simulink library "ammclib_bam_S32K3xx"  (R2016a)
(part 25 of 50)

      |   if (wksi<=0)
      |     warning('Current loop attenuation must be positive.');
      |   end
      |   if (wksi>1)
      |     warning('Current loop attenuation must not exceed 1.');
      |   end
      |   if (J<=0)
      |     warning('Moment of inertia J must be positive.');
      |   end
      |   if (Kt<=0)
      |     warning('Torque constant Kt must be positive.');
      |   end
      |   if (lambdaW<0)
      |     warning('MA filter smoothing factor must be in the range 0..1.');
      |   end
      |   if (lambdaW>1)
      |     warning('MA filter smoothing factor must be in the range 0..1.');
      |   end
      |   if (lambdaFW<0)
      |     warning('MA filter smoothing factor must be in the range 0..1.');
      |   end
      |   if (lambdaFW>1)
      |     warning('MA filter smoothing factor must be in the range 0..1.');
      |   end
      |   if (udcbus<=0)
      |     warning('DC bus voltage must be positive.');
      |   end
      |   if (imax<=0)
      |     warning('Max. phase current must be positive.');
      |   end
      |   if (mechspeed<=0)
      |     warning('Max. speed must be positive.');
      |   end
      |   if (polepairs<1)
      |     warning('Number of pole pairs must be a natural number (1, 2, 3, ...).');
      |   end
      |   if (round(polepairs)~=polepairs)
      |     warning('Number of pole pairs must be a natural number (1, 2, 3, ...).');
      |   end
      |   w0=6.283185307179586*wf0;
      |   pgain=2.0*wksi*w0*J/Kt;
      |   igain=w0*w0*J/Kt;
      |   wmax=polepairs*mechspeed*0.1047197551196598;
      |   fltPropGainQ=pgain;
      |   fltIntegGainQ=igain*SampleTime*0.5;
      |   fltLowerLimitQ=-wmax;
      |   fltUpperLimitQ=wmax;
      |   fltPropGainFW=0.9*pgain;
      |   fltIntegGainFW=fltIntegGainQ;
      |   if (Idmax<0)
      |     iratio=Idmax/imax;
      |     iratio=abs(iratio);
      |     if (abs(iratio) > 1)
      |       iratio = 0;
      |     end
      |     lowlim=acos(iratio)-1.570796326794897;
      |   else
      |     lowlim=0.0;
      |   end
      |   fltLowerLimitFW=lowlim;
      |   fltUpperLimitFW=0.0;
      |   fltLambdaW=lambdaW;
      |   fltLambdaFW=lambdaFW;
      |   rampsc=polepairs*abs(ramprpm)*0.1047197551196598;
      |   fltRampUp=rampsc;
      |   fltRampDown=rampsc;
      |   fltUmaxDivImax=0.5773502691896258*udcbus/imax;
      |   if isnan(fltUmaxDivImax)
      |     if ~strcmp(fltUmaxDivImax_bkup,'0')
      |       set_param(gcb,'fltUmaxDivImax','0');
      |     end
      |   else
      |     tmps=num2str(fltUmaxDivImax);
      |     if ~strcmp(fltUmaxDivImax_bkup,tmps)
      |       set_param(gcb,'fltUmaxDivImax',tmps);
      |     end
      |   end
      |   if isnan(fltLambdaW)
      |     if ~strcmp(fltLambdaW_bkup,'0')
      |       set_param(gcb,'fltLambdaW','0');
      |     end
      |   else
      |     tmps=num2str(fltLambdaW);
      |     if ~strcmp(fltLambdaW_bkup,tmps)
      |       set_param(gcb,'fltLambdaW',tmps);
      |     end
      |   end
      |   if isnan(fltLambdaFW)
      |     if ~strcmp(fltLambdaFW_bkup,'0')
      |       set_param(gcb,'fltLambdaFW','0');
      |     end
      |   else
      |     tmps=num2str(fltLambdaFW);
      |     if ~strcmp(fltLambdaFW_bkup,tmps)
      |       set_param(gcb,'fltLambdaFW',tmps);
      |     end
      |   end
      |   if isnan(fltPropGainQ)
      |     if ~strcmp(fltPropGainQ_bkup,'0')
      |       set_param(gcb,'fltPropGainQ','0');
      |     end
      |   else
      |     tmps=num2str(fltPropGainQ);
      |     if ~strcmp(fltPropGainQ_bkup,tmps)
      |       set_param(gcb,'fltPropGainQ',tmps);
      |     end
      |   end
      |   if isnan(fltIntegGainQ)
      |     if ~strcmp(fltIntegGainQ_bkup,'0')
      |       set_param(gcb,'fltIntegGainQ','0');
      |     end
      |   else
      |     tmps=num2str(fltIntegGainQ);
      |     if ~strcmp(fltIntegGainQ_bkup,tmps)
      |       set_param(gcb,'fltIntegGainQ',tmps);
      |     end
      |   end
      |   if isnan(fltLowerLimitQ)
      |     if ~strcmp(fltLowerLimitQ_bkup,'0')
      |       set_param(gcb,'fltLowerLimitQ','0');
      |     end
      |   else
      |     tmps=num2str(fltLowerLimitQ);
      |     if ~strcmp(fltLowerLimitQ_bkup,tmps)
      |       set_param(gcb,'fltLowerLimitQ',tmps);
      |     end
      |   end
      |   if isnan(fltUpperLimitQ)
      |     if ~strcmp(fltUpperLimitQ_bkup,'0')
      |       set_param(gcb,'fltUpperLimitQ','0');
      |     end
      |   else
      |     tmps=num2str(fltUpperLimitQ);
      |     if ~strcmp(fltUpperLimitQ_bkup,tmps)
      |       set_param(gcb,'fltUpperLimitQ',tmps);
      |     end
      |   end
      |   if isnan(fltPropGainFW)
      |     if ~strcmp(fltPropGainFW_bkup,'0')
      |       set_param(gcb,'fltPropGainFW','0');
      |     end
      |   else
      |     tmps=num2str(fltPropGainFW);
      |     if ~strcmp(fltPropGainFW_bkup,tmps)
      |       set_param(gcb,'fltPropGainFW',tmps);
      |     end
      |   end
      |   if isnan(fltIntegGainFW)
      |     if ~strcmp(fltIntegGainFW_bkup,'0')
      |       set_param(gcb,'fltIntegGainFW','0');
      |     end
      |   else
      |     tmps=num2str(fltIntegGainFW);
      |     if ~strcmp(fltIntegGainFW_bkup,tmps)
      |       set_param(gcb,'fltIntegGainFW',tmps);
      |     end
      |   end
      |   if isnan(fltLowerLimitFW)
      |     if ~strcmp(fltLowerLimitFW_bkup,'0')
      |       set_param(gcb,'fltLowerLimitFW','0');
      |     end
      |   else
      |     tmps=num2str(fltLowerLimitFW);
      |     if ~strcmp(fltLowerLimitFW_bkup,tmps)
      |       set_param(gcb,'fltLowerLimitFW',tmps);
      |     end
      |   end
      |   if isnan(fltUpperLimitFW)
      |     if ~strcmp(fltUpperLimitFW_bkup,'0')
      |       set_param(gcb,'fltUpperLimitFW','0');
      |     end
      |   else
      |     tmps=num2str(fltUpperLimitFW);
      |     if ~strcmp(fltUpperLimitFW_bkup,tmps)
      |       set_param(gcb,'fltUpperLimitFW',tmps);
      |     end
      |   end
      |   if isnan(fltRampUp)
      |     if ~strcmp(fltRampUp_bkup,'0')
      |       set_param(gcb,'fltRampUp','0');
      |     end
      |   else
      |     tmps=num2str(fltRampUp);
      |     if ~strcmp(fltRampUp_bkup,tmps)
      |       set_param(gcb,'fltRampUp',tmps);
      |     end
      |   end
      |   if isnan(fltRampDown)
      |     if ~strcmp(fltRampDown_bkup,'0')
      |       set_param(gcb,'fltRampDown','0');
      |     end
      |   else
      |     tmps=num2str(fltRampDown);
      |     if ~strcmp(fltRampDown_bkup,tmps)
      |       set_param(gcb,'fltRampDown',tmps);
      |     end
      |   end
      | end
      mask Callback polepairs:
      | autoCalcEn=get_param(gcb,'autoCalcEn');
      | if strcmp(autoCalcEn,'on')
      |   SampleTime=Simulink.data.evalinGlobal(bdroot,get_param(gcb,'SampleTime'));
      |   if (SampleTime==-1)
      |     SampleTime=str2double(get_param(gcb,'SampleTime_1'));
      |   end
      |   fltUmaxDivImax_bkup=get_param(gcb,'fltUmaxDivImax');
      |   fltLambdaW_bkup=get_param(gcb,'fltLambdaW');
      |   fltLambdaFW_bkup=get_param(gcb,'fltLambdaFW');
      |   fltPropGainQ_bkup=get_param(gcb,'fltPropGainQ');
      |   fltIntegGainQ_bkup=get_param(gcb,'fltIntegGainQ');
      |   fltLowerLimitQ_bkup=get_param(gcb,'fltLowerLimitQ');
      |   fltUpperLimitQ_bkup=get_param(gcb,'fltUpperLimitQ');
      |   fltPropGainFW_bkup=get_param(gcb,'fltPropGainFW');
      |   fltIntegGainFW_bkup=get_param(gcb,'fltIntegGainFW');
      |   fltLowerLimitFW_bkup=get_param(gcb,'fltLowerLimitFW');
      |   fltUpperLimitFW_bkup=get_param(gcb,'fltUpperLimitFW');
      |   fltRampUp_bkup=get_param(gcb,'fltRampUp');
      |   fltRampDown_bkup=get_param(gcb,'fltRampDown');
      |   wf0=Simulink.data.evalinGlobal(bdroot,get_param(gcb,'wf0'));
      |   wksi=Simulink.data.evalinGlobal(bdroot,get_param(gcb,'wksi'));
      |   J=Simulink.data.evalinGlobal(bdroot,get_param(gcb,'J'));
      |   Kt=Simulink.data.evalinGlobal(bdroot,get_param(gcb,'Kt'));
      |   lambdaW=Simulink.data.evalinGlobal(bdroot,get_param(gcb,'lambdaW'));
      |   lambdaFW=Simulink.data.evalinGlobal(bdroot,get_param(gcb,'lambdaFW'));
      |   Idmax=Simulink.data.evalinGlobal(bdroot,get_param(gcb,'Idmax'));
      |   imax=Simulink.data.evalinGlobal(bdroot,get_param(gcb,'imax'));
      |   udcbus=Simulink.data.evalinGlobal(bdroot,get_param(gcb,'udcbus'));
      |   ramprpm=Simulink.data.evalinGlobal(bdroot,get_param(gcb,'ramprpm'));
      |   mechspeed=Simulink.data.evalinGlobal(bdroot,get_param(gcb,'mechspeed'));
      |   polepairs=Simulink.data.evalinGlobal(bdroot,get_param(gcb,'polepairs'));
      |   if (wf0<=0)
      |     warning('Natural frequency f0 must be positive.');
      |   end
      |   if (wksi<=0)
      |     warning('Current loop attenuation must be positive.');
      |   end
      |   if (wksi>1)
      |     warning('Current loop attenuation must not exceed 1.');
      |   end
      |   if (J<=0)
      |     warning('Moment of inertia J must be positive.');
      |   end
      |   if (Kt<=0)
      |     warning('Torque constant Kt must be positive.');
      |   end
      |   if (lambdaW<0)
      |     warning('MA filter smoothing factor must be in the range 0..1.');
      |   end
      |   if (lambdaW>1)
      |     warning('MA filter smoothing factor must be in the range 0..1.');
      |   end
      |   if (lambdaFW<0)
      |     warning('MA filter smoothing factor must be in the range 0..1.');
      |   end
      |   if (lambdaFW>1)
      |     warning('MA filter smoothing factor must be in the range 0..1.');
      |   end
      |   if (udcbus<=0)
      |     warning('DC bus voltage must be positive.');
      |   end
      |   if (imax<=0)
      |     warning('Max. phase current must be positive.');
      |   end
      |   if (mechspeed<=0)
      |     warning('Max. speed must be positive.');
      |   end
      |   if (polepairs<1)
      |     warning('Number of pole pairs must be a natural number (1, 2, 3, ...).');
      |   end
      |   if (round(polepairs)~=polepairs)
      |     warning('Number of pole pairs must be a natural number (1, 2, 3, ...).');
      |   end
      |   w0=6.283185307179586*wf0;
      |   pgain=2.0*wksi*w0*J/Kt;
      |   igain=w0*w0*J/Kt;
      |   wmax=polepairs*mechspeed*0.1047197551196598;
      |   fltPropGainQ=pgain;
      |   fltIntegGainQ=igain*SampleTime*0.5;
      |   fltLowerLimitQ=-wmax;
      |   fltUpperLimitQ=wmax;
      |   fltPropGainFW=0.9*pgain;
      |   fltIntegGainFW=fltIntegGainQ;
      |   if (Idmax<0)
      |     iratio=Idmax/imax;
      |     iratio=abs(iratio);
      |     if (abs(iratio) > 1)
      |       iratio = 0;
      |     end
      |     lowlim=acos(iratio)-1.570796326794897;
      |   else
      |     lowlim=0.0;
      |   end
      |   fltLowerLimitFW=lowlim;
      |   fltUpperLimitFW=0.0;
      |   fltLambdaW=lambdaW;
      |   fltLambdaFW=lambdaFW;
      |   rampsc=polepairs*abs(ramprpm)*0.1047197551196598;
      |   fltRampUp=rampsc;
      |   fltRampDown=rampsc;
      |   fltUmaxDivImax=0.5773502691896258*udcbus/imax;
      |   if isnan(fltUmaxDivImax)
      |     if ~strcmp(fltUmaxDivImax_bkup,'0')
      |       set_param(gcb,'fltUmaxDivImax','0');
      |     end
      |   else
      |     tmps=num2str(fltUmaxDivImax);
      |     if ~strcmp(fltUmaxDivImax_bkup,tmps)
      |       set_param(gcb,'fltUmaxDivImax',tmps);
      |     end
      |   end
      |   if isnan(fltLambdaW)
      |     if ~strcmp(fltLambdaW_bkup,'0')
      |       set_param(gcb,'fltLambdaW','0');
      |     end
      |   else
      |     tmps=num2str(fltLambdaW);
      |     if ~strcmp(fltLambdaW_bkup,tmps)
      |       set_param(gcb,'fltLambdaW',tmps);
      |     end
      |   end
      |   if isnan(fltLambdaFW)
      |     if ~strcmp(fltLambdaFW_bkup,'0')
      |       set_param(gcb,'fltLambdaFW','0');
      |     end
      |   else
      |     tmps=num2str(fltLambdaFW);
      |     if ~strcmp(fltLambdaFW_bkup,tmps)
      |       set_param(gcb,'fltLambdaFW',tmps);
      |     end
      |   end
      |   if isnan(fltPropGainQ)
      |     if ~strcmp(fltPropGainQ_bkup,'0')
      |       set_param(gcb,'fltPropGainQ','0');
      |     end
      |   else
      |     tmps=num2str(fltPropGainQ);
      |     if ~strcmp(fltPropGainQ_bkup,tmps)
      |       set_param(gcb,'fltPropGainQ',tmps);
      |     end
      |   end
      |   if isnan(fltIntegGainQ)
      |     if ~strcmp(fltIntegGainQ_bkup,'0')
      |       set_param(gcb,'fltIntegGainQ','0');
      |     end
      |   else
      |     tmps=num2str(fltIntegGainQ);
      |     if ~strcmp(fltIntegGainQ_bkup,tmps)
      |       set_param(gcb,'fltIntegGainQ',tmps);
      |     end
      |   end
      |   if isnan(fltLowerLimitQ)
      |     if ~strcmp(fltLowerLimitQ_bkup,'0')
      |       set_param(gcb,'fltLowerLimitQ','0');
      |     end
      |   else
      |     tmps=num2str(fltLowerLimitQ);
      |     if ~strcmp(fltLowerLimitQ_bkup,tmps)
      |       set_param(gcb,'fltLowerLimitQ',tmps);
      |     end
      |   end
      |   if isnan(fltUpperLimitQ)
      |     if ~strcmp(fltUpperLimitQ_bkup,'0')
      |       set_param(gcb,'fltUpperLimitQ','0');
      |     end
      |   else
      |     tmps=num2str(fltUpperLimitQ);
      |     if ~strcmp(fltUpperLimitQ_bkup,tmps)
      |       set_param(gcb,'fltUpperLimitQ',tmps);
      |     end
      |   end
      |   if isnan(fltPropGainFW)
      |     if ~strcmp(fltPropGainFW_bkup,'0')
      |       set_param(gcb,'fltPropGainFW','0');
      |     end
      |   else
      |     tmps=num2str(fltPropGainFW);
      |     if ~strcmp(fltPropGainFW_bkup,tmps)
      |       set_param(gcb,'fltPropGainFW',tmps);
      |     end
      |   end
      |   if isnan(fltIntegGainFW)
      |     if ~strcmp(fltIntegGainFW_bkup,'0')
      |       set_param(gcb,'fltIntegGainFW','0');
      |     end
      |   else
      |     tmps=num2str(fltIntegGainFW);
      |     if ~strcmp(fltIntegGainFW_bkup,tmps)
      |       set_param(gcb,'fltIntegGainFW',tmps);
      |     end
      |   end
      |   if isnan(fltLowerLimitFW)
      |     if ~strcmp(fltLowerLimitFW_bkup,'0')
      |       set_param(gcb,'fltLowerLimitFW','0');
      |     end
      |   else
      |     tmps=num2str(fltLowerLimitFW);
      |     if ~strcmp(fltLowerLimitFW_bkup,tmps)
      |       set_param(gcb,'fltLowerLimitFW',tmps);
      |     end
      |   end
      |   if isnan(fltUpperLimitFW)
      |     if ~strcmp(fltUpperLimitFW_bkup,'0')
      |       set_param(gcb,'fltUpperLimitFW','0');
      |     end
      |   else
      |     tmps=num2str(fltUpperLimitFW);
      |     if ~strcmp(fltUpperLimitFW_bkup,tmps)
      |       set_param(gcb,'fltUpperLimitFW',tmps);
      |     end
      |   end
      |   if isnan(fltRampUp)
      |     if ~strcmp(fltRampUp_bkup,'0')
      |       set_param(gcb,'fltRampUp','0');
      |     end
      |   else
      |     tmps=num2str(fltRampUp);
      |     if ~strcmp(fltRampUp_bkup,tmps)
      |       set_param(gcb,'fltRampUp',tmps);
      |     end
      |   end
      |   if isnan(fltRampDown)
      |     if ~strcmp(fltRampDown_bkup,'0')
      |       set_param(gcb,'fltRampDown','0');
      |     end
      |   else
      |     tmps=num2str(fltRampDown);
      |     if ~strcmp(fltRampDown_bkup,tmps)
      |       set_param(gcb,'fltRampDown',tmps);
      |     end
      |   end
      | end
      mask Callback autoCalcEn:
      | maskStr=get_param(gcb,'showStates');
      | if strcmp(maskStr,'Hide (faster execution)')
      |   p=Simulink.Mask.get(gcb);
      |   autoCalcEn=get_param(gcb,'autoCalcEn');
      |   hintText=p.getDialogControl('timeHint');
      |   if strcmp(autoCalcEn,'on')
      |     param=p.getParameter('polepairs');
      |     if strcmp(param.Enabled,'off')
      |       SampleTime=Simulink.data.evalinGlobal(bdroot,get_param(gcb,'SampleTime'));
      |       if SampleTime==-1
      |         SampleTime=str2double(get_param(gcb,'SampleTime_1'));
      |         if isnan(SampleTime)
      |           hintText.Prompt=['Note: Implementation parameters cannot be calculated yet because the block''s inherited sample time is unknown. Simulink will update the sample time when you run the simulation.'];
      |         else
      |           hintText.Prompt=['Caution: Implementation parameters depend on inherited sample time. Make sure that the sample time of the block''s inputs corresponds to the sampling period in the target application.'];
      |         end
      |       else
      |         hintText.Prompt='Caution: Implementation parameters depend on the sample time. Make sure that the simulation time step corresponds to the sampling period in the target application.';
      |       end
      |       p=Simulink.Mask.get(gcb);
      |       param=p.getParameter('wf0');
      |       param.set('Enabled','on');
      |       param=p.getParameter('wksi');
      |       param.set('Enabled','on');
      |       param=p.getParameter('J');
      |       param.set('Enabled','on');
      |       param=p.getParameter('Kt');
      |       param.set('Enabled','on');
      |       param=p.getParameter('lambdaW');
      |       param.set('Enabled','on');
      |       param=p.getParameter('lambdaFW');
      |       param.set('Enabled','on');
      |       param=p.getParameter('Idmax');
      |       param.set('Enabled','on');
      |       param=p.getParameter('imax');
      |       param.set('Enabled','on');
      |       param=p.getParameter('udcbus');
      |       param.set('Enabled','on');
      |       param=p.getParameter('ramprpm');
      |       param.set('Enabled','on');
      |       param=p.getParameter('mechspeed');
      |       param.set('Enabled','on');
      |       param=p.getParameter('polepairs');
      |       param.set('Enabled','on');
      |     else
      |       SampleTime=Simulink.data.evalinGlobal(bdroot,get_param(gcb,'SampleTime'));
      |       if SampleTime==-1
      |         SampleTime=str2double(get_param(gcb,'SampleTime_1'));
      |       end
      |     end
      |     fltUmaxDivImax_bkup=get_param(gcb,'fltUmaxDivImax');
      |     fltLambdaW_bkup=get_param(gcb,'fltLambdaW');
      |     fltLambdaFW_bkup=get_param(gcb,'fltLambdaFW');
      |     fltPropGainQ_bkup=get_param(gcb,'fltPropGainQ');
      |     fltIntegGainQ_bkup=get_param(gcb,'fltIntegGainQ');
      |     fltLowerLimitQ_bkup=get_param(gcb,'fltLowerLimitQ');
      |     fltUpperLimitQ_bkup=get_param(gcb,'fltUpperLimitQ');
      |     fltPropGainFW_bkup=get_param(gcb,'fltPropGainFW');
      |     fltIntegGainFW_bkup=get_param(gcb,'fltIntegGainFW');
      |     fltLowerLimitFW_bkup=get_param(gcb,'fltLowerLimitFW');
      |     fltUpperLimitFW_bkup=get_param(gcb,'fltUpperLimitFW');
      |     fltRampUp_bkup=get_param(gcb,'fltRampUp');
      |     fltRampDown_bkup=get_param(gcb,'fltRampDown');
      |     wf0=Simulink.data.evalinGlobal(bdroot,get_param(gcb,'wf0'));
      |     wksi=Simulink.data.evalinGlobal(bdroot,get_param(gcb,'wksi'));
      |     J=Simulink.data.evalinGlobal(bdroot,get_param(gcb,'J'));
      |     Kt=Simulink.data.evalinGlobal(bdroot,get_param(gcb,'Kt'));
      |     lambdaW=Simulink.data.evalinGlobal(bdroot,get_param(gcb,'lambdaW'));
      |     lambdaFW=Simulink.data.evalinGlobal(bdroot,get_param(gcb,'lambdaFW'));
      |     Idmax=Simulink.data.evalinGlobal(bdroot,get_param(gcb,'Idmax'));
      |     imax=Simulink.data.evalinGlobal(bdroot,get_param(gcb,'imax'));
      |     udcbus=Simulink.data.evalinGlobal(bdroot,get_param(gcb,'udcbus'));
      |     ramprpm=Simulink.data.evalinGlobal(bdroot,get_param(gcb,'ramprpm'));
      |     mechspeed=Simulink.data.evalinGlobal(bdroot,get_param(gcb,'mechspeed'));
      |     polepairs=Simulink.data.evalinGlobal(bdroot,get_param(gcb,'polepairs'));
      |     if (wf0<=0)
      |       warning('Natural frequency f0 must be positive.');
      |     end
      |     if (wksi<=0)
      |       warning('Current loop attenuation must be positive.');
      |     end
      |     if (wksi>1)
      |       warning('Current loop attenuation must not exceed 1.');
      |     end
      |     if (J<=0)
      |       warning('Moment of inertia J must be positive.');
      |     end
      |     if (Kt<=0)
      |       warning('Torque constant Kt must be positive.');
      |     end
      |     if (lambdaW<0)
      |       warning('MA filter smoothing factor must be in the range 0..1.');
      |     end
      |     if (lambdaW>1)
      |       warning('MA filter smoothing factor must be in the range 0..1.');
      |     end
      |     if (lambdaFW<0)
      |       warning('MA filter smoothing factor must be in the range 0..1.');
      |     end
      |     if (lambdaFW>1)
      |       warning('MA filter smoothing factor must be in the range 0..1.');
      |     end
      |     if (udcbus<=0)
      |       warning('DC bus voltage must be positive.');
      |     end
      |     if (imax<=0)
      |       warning('Max. phase current must be positive.');
      |     end
      |     if (mechspeed<=0)
      |       warning('Max. speed must be positive.');
      |     end
      |     if (polepairs<1)
      |       warning('Number of pole pairs must be a natural number (1, 2, 3, ...).');
      |     end
      |     if (round(polepairs)~=polepairs)
      |       warning('Number of pole pairs must be a natural number (1, 2, 3, ...).');
      |     end
      |     w0=6.283185307179586*wf0;
      |     pgain=2.0*wksi*w0*J/Kt;
      |     igain=w0*w0*J/Kt;
      |     wmax=polepairs*mechspeed*0.1047197551196598;
      |     fltPropGainQ=pgain;
      |     fltIntegGainQ=igain*SampleTime*0.5;
      |     fltLowerLimitQ=-wmax;
      |     fltUpperLimitQ=wmax;
      |     fltPropGainFW=0.9*pgain;
      |     fltIntegGainFW=fltIntegGainQ;
      |     if (Idmax<0)
      |       iratio=Idmax/imax;
      |       iratio=abs(iratio);
      |       if (abs(iratio) > 1)
      |         iratio = 0;
      |       end
      |       lowlim=acos(iratio)-1.570796326794897;
      |     else
      |       lowlim=0.0;
      |     end
      |     fltLowerLimitFW=lowlim;
      |     fltUpperLimitFW=0.0;
      |     fltLambdaW=lambdaW;
      |     fltLambdaFW=lambdaFW;
      |     rampsc=polepairs*abs(ramprpm)*0.1047197551196598;
      |     fltRampUp=rampsc;
      |     fltRampDown=rampsc;
      |     fltUmaxDivImax=0.5773502691896258*udcbus/imax;
      |     if isnan(fltUmaxDivImax)
      |       if ~strcmp(fltUmaxDivImax_bkup,'0')
      |         set_param(gcb,'fltUmaxDivImax','0');
      |       end
      |     else
      |       tmps=num2str(fltUmaxDivImax);
      |       if ~strcmp(fltUmaxDivImax_bkup,tmps)
      |         set_param(gcb,'fltUmaxDivImax',tmps);
      |       end
      |     end
      |     if isnan(fltLambdaW)
      |       if ~strcmp(fltLambdaW_bkup,'0')
      |         set_param(gcb,'fltLambdaW','0');
      |       end
      |     else
      |       tmps=num2str(fltLambdaW);
      |       if ~strcmp(fltLambdaW_bkup,tmps)
      |         set_param(gcb,'fltLambdaW',tmps);
      |       end
      |     end
      |     if isnan(fltLambdaFW)
      |       if ~strcmp(fltLambdaFW_bkup,'0')
      |         set_param(gcb,'fltLambdaFW','0');
      |       end
      |     else
      |       tmps=num2str(fltLambdaFW);
      |       if ~strcmp(fltLambdaFW_bkup,tmps)
      |         set_param(gcb,'fltLambdaFW',tmps);
      |       end
      |     end
      |     if isnan(fltPropGainQ)
      |       if ~strcmp(fltPropGainQ_bkup,'0')
      |         set_param(gcb,'fltPropGainQ','0');
      |       end
      |     else
      |       tmps=num2str(fltPropGainQ);
      |       if ~strcmp(fltPropGainQ_bkup,tmps)
      |         set_param(gcb,'fltPropGainQ',tmps);
      |       end
      |     end
      |     if isnan(fltIntegGainQ)
      |       if ~strcmp(fltIntegGainQ_bkup,'0')
      |         set_param(gcb,'fltIntegGainQ','0');
      |       end
      |     else
      |       tmps=num2str(fltIntegGainQ);
      |       if ~strcmp(fltIntegGainQ_bkup,tmps)
      |         set_param(gcb,'fltIntegGainQ',tmps);
      |       end
      |     end
      |     if isnan(fltLowerLimitQ)
      |       if ~strcmp(fltLowerLimitQ_bkup,'0')
      |         set_param(gcb,'fltLowerLimitQ','0');
      |       end
      |     else
      |       tmps=num2str(fltLowerLimitQ);
      |       if ~strcmp(fltLowerLimitQ_bkup,tmps)
      |         set_param(gcb,'fltLowerLimitQ',tmps);
      |       end
      |     end
      |     if isnan(fltUpperLimitQ)
      |       if ~strcmp(fltUpperLimitQ_bkup,'0')
      |         set_param(gcb,'fltUpperLimitQ','0');
      |       end
      |     else
      |       tmps=num2str(fltUpperLimitQ);
      |       if ~strcmp(fltUpperLimitQ_bkup,tmps)
      |         set_param(gcb,'fltUpperLimitQ',tmps);
      |       end
      |     end
      |     if isnan(fltPropGainFW)
      |       if ~strcmp(fltPropGainFW_bkup,'0')
      |         set_param(gcb,'fltPropGainFW','0');
      |       end
      |     else
      |       tmps=num2str(fltPropGainFW);
      |       if ~strcmp(fltPropGainFW_bkup,tmps)
      |         set_param(gcb,'fltPropGainFW',tmps);
      |       end
      |     end
      |     if isnan(fltIntegGainFW)
      |       if ~strcmp(fltIntegGainFW_bkup,'0')
      |         set_param(gcb,'fltIntegGainFW','0');
      |       end
      |     else
      |       tmps=num2str(fltIntegGainFW);
      |       if ~strcmp(fltIntegGainFW_bkup,tmps)
      |         set_param(gcb,'fltIntegGainFW',tmps);
      |       end
      |     end
      |     if isnan(fltLowerLimitFW)
      |       if ~strcmp(fltLowerLimitFW_bkup,'0')
      |         set_param(gcb,'fltLowerLimitFW','0');
      |       end
      |     else
      |       tmps=num2str(fltLowerLimitFW);
      |       if ~strcmp(fltLowerLimitFW_bkup,tmps)
      |         set_param(gcb,'fltLowerLimitFW',tmps);
      |       end
      |     end
      |     if isnan(fltUpperLimitFW)
      |       if ~strcmp(fltUpperLimitFW_bkup,'0')
      |         set_param(gcb,'fltUpperLimitFW','0');
      |       end
      |     else
      |       tmps=num2str(fltUpperLimitFW);
      |       if ~strcmp(fltUpperLimitFW_bkup,tmps)
      |         set_param(gcb,'fltUpperLimitFW',tmps);
      |       end
      |     end
      |     if isnan(fltRampUp)
      |       if ~strcmp(fltRampUp_bkup,'0')
      |         set_param(gcb,'fltRampUp','0');
      |       end
      |     else
      |       tmps=num2str(fltRampUp);
      |       if ~strcmp(fltRampUp_bkup,tmps)
      |         set_param(gcb,'fltRampUp',tmps);
      |       end
      |     end
      |     if isnan(fltRampDown)
      |       if ~strcmp(fltRampDown_bkup,'0')
      |         set_param(gcb,'fltRampDown','0');
      |       end
      |     else
      |       tmps=num2str(fltRampDown);
      |       if ~strcmp(fltRampDown_bkup,tmps)
      |         set_param(gcb,'fltRampDown',tmps);
      |       end
      |     end
      |   else
      |     param=p.getParameter('polepairs');
      |     if strcmp(param.Enabled,'on')
      |       hintText.Prompt='Caution: Implementation parameters are fixed.';
      |       p=Simulink.Mask.get(gcb);
      |       param=p.getParameter('wf0');
      |       param.set('Enabled','off');
      |       param=p.getParameter('wksi');
      |       param.set('Enabled','off');
      |       param=p.getParameter('J');
      |       param.set('Enabled','off');
      |       param=p.getParameter('Kt');
      |       param.set('Enabled','off');
      |       param=p.getParameter('lambdaW');
      |       param.set('Enabled','off');
      |       param=p.getParameter('lambdaFW');
      |       param.set('Enabled','off');
      |       param=p.getParameter('Idmax');
      |       param.set('Enabled','off');
      |       param=p.getParameter('imax');
      |       param.set('Enabled','off');
      |       param=p.getParameter('udcbus');
      |       param.set('Enabled','off');
      |       param=p.getParameter('ramprpm');
      |       param.set('Enabled','off');
      |       param=p.getParameter('mechspeed');
      |       param.set('Enabled','off');
      |       param=p.getParameter('polepairs');
      |       param.set('Enabled','off');
      |     end
      |   end
      | end
      mask DialogControl CompBut Prompt: Recalculate sample times
      mask DialogControl CompBut Tooltip: Simulink updates the sample times of all blocks when the simulation is run. This button will update the sample times now.
      mask DialogControl CompBut Callback:
      | btn=questdlg('This will apply all changes in all open dialog boxes and update the schematic. Do you want to proceed?','Apply all changes','Continue','Cancel','Continue');
      | if strcmp(btn,'Continue')
      |   dlgs=DAStudio.ToolRoot.getOpenDialogs;
      |   for i=1:length(dlgs)
      |     dlgs(i).apply;
      |   end
      |   try
      |     SampleTime_1=str2double(get_param(gcb,'SampleTime_1'));
      |     ts=Simulink.Block.getSampleTimes(gcb);
      |     ts=ts(1).Value(1);
      |     if (SampleTime_1 ~= ts)
      |       SampleTime_1=ts;
      |       set_param(gcb,'SampleTime_1',num2str(ts));
      |       autoCalcEn=get_param(gcb,'autoCalcEn');
      |       if strcmp(autoCalcEn,'on')
      |         SampleTime=Simulink.data.evalinGlobal(bdroot,get_param(gcb,'SampleTime'));
      |         p=Simulink.Mask.get(gcb);
      |         hintText=p.getDialogControl('timeHint');
      |         if SampleTime==-1
      |           SampleTime=SampleTime_1;
      |           hintText.Prompt='Caution: Implementation parameters depend on inherited sample time. Make sure that the sample time of the block''s inputs corresponds to the sampling period in the target application.';
      |         else
      |           hintText.Prompt='Caution: Implementation parameters depend on the sample time. Make sure that the simulation time step corresponds to the sampling period in the target application.';
      |         end
      |         fltUmaxDivImax_bkup=get_param(gcb,'fltUmaxDivImax');
      |         fltLambdaW_bkup=get_param(gcb,'fltLambdaW');
      |         fltLambdaFW_bkup=get_param(gcb,'fltLambdaFW');
      |         fltPropGainQ_bkup=get_param(gcb,'fltPropGainQ');
      |         fltIntegGainQ_bkup=get_param(gcb,'fltIntegGainQ');
      |         fltLowerLimitQ_bkup=get_param(gcb,'fltLowerLimitQ');
      |         fltUpperLimitQ_bkup=get_param(gcb,'fltUpperLimitQ');
      |         fltPropGainFW_bkup=get_param(gcb,'fltPropGainFW');
      |         fltIntegGainFW_bkup=get_param(gcb,'fltIntegGainFW');
      |         fltLowerLimitFW_bkup=get_param(gcb,'fltLowerLimitFW');
      |         fltUpperLimitFW_bkup=get_param(gcb,'fltUpperLimitFW');
      |         fltRampUp_bkup=get_param(gcb,'fltRampUp');
      |         fltRampDown_bkup=get_param(gcb,'fltRampDown');
      |         wf0=Simulink.data.evalinGlobal(bdroot,get_param(gcb,'wf0'));
      |         wksi=Simulink.data.evalinGlobal(bdroot,get_param(gcb,'wksi'));
      |         J=Simulink.data.evalinGlobal(bdroot,get_param(gcb,'J'));
      |         Kt=Simulink.data.evalinGlobal(bdroot,get_param(gcb,'Kt'));
      |         lambdaW=Simulink.data.evalinGlobal(bdroot,get_param(gcb,'lambdaW'));
      |         lambdaFW=Simulink.data.evalinGlobal(bdroot,get_param(gcb,'lambdaFW'));
      |         Idmax=Simulink.data.evalinGlobal(bdroot,get_param(gcb,'Idmax'));
      |         imax=Simulink.data.evalinGlobal(bdroot,get_param(gcb,'imax'));
      |         udcbus=Simulink.data.evalinGlobal(bdroot,get_param(gcb,'udcbus'));
      |         ramprpm=Simulink.data.evalinGlobal(bdroot,get_param(gcb,'ramprpm'));
      |         mechspeed=Simulink.data.evalinGlobal(bdroot,get_param(gcb,'mechspeed'));
      |         polepairs=Simulink.data.evalinGlobal(bdroot,get_param(gcb,'polepairs'));
      |         if (wf0<=0)
      |           warning('Natural frequency f0 must be positive.');
      |         end
      |         if (wksi<=0)
      |           warning('Current loop attenuation must be positive.');
      |         end
      |         if (wksi>1)
      |           warning('Current loop attenuation must not exceed 1.');
      |         end
      |         if (J<=0)
      |           warning('Moment of inertia J must be positive.');
      |         end
      |         if (Kt<=0)
      |           warning('Torque constant Kt must be positive.');
      |         end
      |         if (lambdaW<0)
      |           warning('MA filter smoothing factor must be in the range 0..1.');
      |         end
      |         if (lambdaW>1)
      |           warning('MA filter smoothing factor must be in the range 0..1.');
      |         end
      |         if (lambdaFW<0)
      |           warning('MA filter smoothing factor must be in the range 0..1.');
      |         end
      |         if (lambdaFW>1)
      |           warning('MA filter smoothing factor must be in the range 0..1.');
      |         end
      |         if (udcbus<=0)
      |           warning('DC bus voltage must be positive.');
      |         end
      |         if (imax<=0)
      |           warning('Max. phase current must be positive.');
      |         end
      |         if (mechspeed<=0)
      |           warning('Max. speed must be positive.');
      |         end
      |         if (polepairs<1)
      |           warning('Number of pole pairs must be a natural number (1, 2, 3, ...).');
      |         end
      |         if (round(polepairs)~=polepairs)
      |           warning('Number of pole pairs must be a natural number (1, 2, 3, ...).');
      |         end
      |         w0=6.283185307179586*wf0;
      |         pgain=2.0*wksi*w0*J/Kt;
      |         igain=w0*w0*J/Kt;
      |         wmax=polepairs*mechspeed*0.1047197551196598;
      |         fltPropGainQ=pgain;
      |         fltIntegGainQ=igain*SampleTime*0.5;
      |         fltLowerLimitQ=-wmax;
      |         fltUpperLimitQ=wmax;
      |         fltPropGainFW=0.9*pgain;
      |         fltIntegGainFW=fltIntegGainQ;
      |         if (Idmax<0)
      |           iratio=Idmax/imax;
      |           iratio=abs(iratio);
      |           if (abs(iratio) > 1)
      |             iratio = 0;
      |           end
      |           lowlim=acos(iratio)-1.570796326794897;
      |         else
      |           lowlim=0.0;
      |         end
      |         fltLowerLimitFW=lowlim;
      |         fltUpperLimitFW=0.0;
      |         fltLambdaW=lambdaW;
      |         fltLambdaFW=lambdaFW;
      |         rampsc=polepairs*abs(ramprpm)*0.1047197551196598;
      |         fltRampUp=rampsc;
      |         fltRampDown=rampsc;
      |         fltUmaxDivImax=0.5773502691896258*udcbus/imax;
      |         if isnan(fltUmaxDivImax)
      |           if ~strcmp(fltUmaxDivImax_bkup,'0')
      |             set_param(gcb,'fltUmaxDivImax','0');
      |           end
      |         else
      |           tmps=num2str(fltUmaxDivImax);
      |           if ~strcmp(fltUmaxDivImax_bkup,tmps)
      |             set_param(gcb,'fltUmaxDivImax',tmps);
      |           end
      |         end
      |         if isnan(fltLambdaW)
      |           if ~strcmp(fltLambdaW_bkup,'0')
      |             set_param(gcb,'fltLambdaW','0');
      |           end
      |         else
      |           tmps=num2str(fltLambdaW);
      |           if ~strcmp(fltLambdaW_bkup,tmps)
      |             set_param(gcb,'fltLambdaW',tmps);
      |           end
      |         end
      |         if isnan(fltLambdaFW)
      |           if ~strcmp(fltLambdaFW_bkup,'0')
      |             set_param(gcb,'fltLambdaFW','0');
      |           end
      |         else
      |           tmps=num2str(fltLambdaFW);
      |           if ~strcmp(fltLambdaFW_bkup,tmps)
      |             set_param(gcb,'fltLambdaFW',tmps);
      |           end
      |         end
      |         if isnan(fltPropGainQ)
      |           if ~strcmp(fltPropGainQ_bkup,'0')
      |             set_param(gcb,'fltPropGainQ','0');
      |           end
      |         else
      |           tmps=num2str(fltPropGainQ);
      |           if ~strcmp(fltPropGainQ_bkup,tmps)
      |             set_param(gcb,'fltPropGainQ',tmps);
      |           end
      |         end
      |         if isnan(fltIntegGainQ)
      |           if ~strcmp(fltIntegGainQ_bkup,'0')
      |             set_param(gcb,'fltIntegGainQ','0');
      |           end
      |         else
      |           tmps=num2str(fltIntegGainQ);
      |           if ~strcmp(fltIntegGainQ_bkup,tmps)
      |             set_param(gcb,'fltIntegGainQ',tmps);
      |           end
      |         end
      |         if isnan(fltLowerLimitQ)
      |           if ~strcmp(fltLowerLimitQ_bkup,'0')
      |             set_param(gcb,'fltLowerLimitQ','0');
      |           end
      |         else
      |           tmps=num2str(fltLowerLimitQ);
      |           if ~strcmp(fltLowerLimitQ_bkup,tmps)
      |             set_param(gcb,'fltLowerLimitQ',tmps);
      |           end
      |         end
      |         if isnan(fltUpperLimitQ)
      |           if ~strcmp(fltUpperLimitQ_bkup,'0')
      |             set_param(gcb,'fltUpperLimitQ','0');
      |           end
      |         else
      |           tmps=num2str(fltUpperLimitQ);
      |           if ~strcmp(fltUpperLimitQ_bkup,tmps)
      |             set_param(gcb,'fltUpperLimitQ',tmps);
      |           end
      |         end
      |         if isnan(fltPropGainFW)
      |           if ~strcmp(fltPropGainFW_bkup,'0')
      |             set_param(gcb,'fltPropGainFW','0');
      |           end
      |         else
      |           tmps=num2str(fltPropGainFW);
      |           if ~strcmp(fltPropGainFW_bkup,tmps)
      |             set_param(gcb,'fltPropGainFW',tmps);
      |           end
      |         end
      |         if isnan(fltIntegGainFW)
      |           if ~strcmp(fltIntegGainFW_bkup,'0')
      |             set_param(gcb,'fltIntegGainFW','0');
      |           end
      |         else
      |           tmps=num2str(fltIntegGainFW);
      |           if ~strcmp(fltIntegGainFW_bkup,tmps)
      |             set_param(gcb,'fltIntegGainFW',tmps);
      |           end
      |         end
      |         if isnan(fltLowerLimitFW)
      |           if ~strcmp(fltLowerLimitFW_bkup,'0')
      |             set_param(gcb,'fltLowerLimitFW','0');
      |           end
      |         else
      |           tmps=num2str(fltLowerLimitFW);
      |           if ~strcmp(fltLowerLimitFW_bkup,tmps)
      |             set_param(gcb,'fltLowerLimitFW',tmps);
      |           end
      |         end
      |         if isnan(fltUpperLimitFW)
      |           if ~strcmp(fltUpperLimitFW_bkup,'0')
      |             set_param(gcb,'fltUpperLimitFW','0');
      |           end
      |         else
      |           tmps=num2str(fltUpperLimitFW);
      |           if ~strcmp(fltUpperLimitFW_bkup,tmps)
      |             set_param(gcb,'fltUpperLimitFW',tmps);
      |           end
      |         end
      |         if isnan(fltRampUp)
      |           if ~strcmp(fltRampUp_bkup,'0')
      |             set_param(gcb,'fltRampUp','0');
      |           end
      |         else
      |           tmps=num2str(fltRampUp);
      |           if ~strcmp(fltRampUp_bkup,tmps)
      |             set_param(gcb,'fltRampUp',tmps);
      |           end
      |         end
      |         if isnan(fltRampDown)
      |           if ~strcmp(fltRampDown_bkup,'0')
      |             set_param(gcb,'fltRampDown','0');
      |           end
      |         else
      |           tmps=num2str(fltRampDown);
      |           if ~strcmp(fltRampDown_bkup,tmps)
      |             set_param(gcb,'fltRampDown',tmps);
      |           end
      |         end
      |       end
      |     end
      |   catch
      |    warning(['Sample time cannot be calculated for the block ' gcb])
      |   end
      | end
      mask DialogControl timeHint Prompt: Note: Implementation parameters cannot be calculated yet because the block's inherited sample time is unknown. Simulink will update the sample time when you run the simulation.
      mask Display:
      | color('black');
      | pos = get_param(gcb, 'Position');
      | width = pos(3) - pos(1);
      | height = pos(4) - pos(2);
      | tX=width/2;
      | tY=height - 25;
      | color('black');
      | text(tX,tY, 'AMCLIB_FWSpeedLoop_FLT', 'horizontalAlignment', 'center');
      | if showStates == 2
      |   color('red');
      |   text(tX,tY - 20, ['debugging mode' char(13) char(10) '(limited performance)'], 'horizontalAlignment', 'center');
      | end
  AMCLIB_FW_FLT : Subsystem  StartFcn=|  TreatAsAtomicUnit=on  mask(AMCLIB_FW_FLT){showStates=Hide (faster execution), resetStatesEnable=Pre-set according to the first set of inputs after reset, showDebugOutputs=Hide, SampleTime=-1, wf0=30, wksi=1, J=1.6e-5, Kt=0.067, lambdaFW=0.9, Idmax=-5, imax=10, udcbus=12, autoCalcEn=on, fltUmaxDivImax=0, fltLambda=0, fltPropGain=0, fltIntegGain=0, fltLowerLimit=0, fltUpperLimit=0, SampleTime_1=NaN}
      | ts=get_param(gcb,'CompiledSampleTime');
      | if iscell(ts)
      |   ts=ts{1};
      |   if iscell(ts)
      |     ts=ts{1};
      |   end
      | end
      | ts=ts(1);
      | set_param(gcb,'SampleTime_1',num2str(ts));
      | p=Simulink.Mask.get(gcb);
      | hintText=p.getDialogControl('timeHint');
      | SampleTime=Simulink.data.evalinGlobal(bdroot,get_param(gcb,'SampleTime'));
      | p=Simulink.Mask.get(gcb);
      | autoCalcEn=get_param(gcb,'autoCalcEn');
      | if strcmp(autoCalcEn,'on')
      |   if SampleTime==-1
      |     hintText.Prompt='Caution: Implementation parameters depend on inherited sample time. Make sure that the sample time of the block''s inputs corresponds to the sampling period in the target application.';
      |   else
      |     hintText.Prompt='Caution: Implementation parameters depend on the sample time. Make sure that the simulation time step corresponds to the sampling period in the target application.';
      |   end
      |   SampleTime=ts;
      |   fltUmaxDivImax_bkup=get_param(gcb,'fltUmaxDivImax');
      |   fltLambda_bkup=get_param(gcb,'fltLambda');
      |   fltPropGain_bkup=get_param(gcb,'fltPropGain');
      |   fltIntegGain_bkup=get_param(gcb,'fltIntegGain');
      |   fltLowerLimit_bkup=get_param(gcb,'fltLowerLimit');
      |   fltUpperLimit_bkup=get_param(gcb,'fltUpperLimit');
      |   wf0=Simulink.data.evalinGlobal(bdroot,get_param(gcb,'wf0'));
      |   wksi=Simulink.data.evalinGlobal(bdroot,get_param(gcb,'wksi'));
      |   J=Simulink.data.evalinGlobal(bdroot,get_param(gcb,'J'));
      |   Kt=Simulink.data.evalinGlobal(bdroot,get_param(gcb,'Kt'));
      |   lambdaFW=Simulink.data.evalinGlobal(bdroot,get_param(gcb,'lambdaFW'));
      |   Idmax=Simulink.data.evalinGlobal(bdroot,get_param(gcb,'Idmax'));
      |   imax=Simulink.data.evalinGlobal(bdroot,get_param(gcb,'imax'));
      |   udcbus=Simulink.data.evalinGlobal(bdroot,get_param(gcb,'udcbus'));
      |   if (wf0<=0)
      |     warning('Natural frequency f0 must be positive.');
      |   end
      |   if (wksi<=0)
      |     warning('Current loop attenuation must be positive.');
      |   end
      |   if (wksi>1)
      |     warning('Current loop attenuation must not exceed 1.');
      |   end
      |   if (J<=0)
      |     warning('Moment of inertia J must be positive.');
      |   end
      |   if (Kt<=0)
      |     warning('Torque constant Kt must be positive.');
      |   end
      |   if (lambdaFW<0)
      |     warning('MA filter smoothing factor must be in the range 0..1.');
      |   end
      |   if (lambdaFW>1)
      |     warning('MA filter smoothing factor must be in the range 0..1.');
      |   end
      |   if (udcbus<=0)
      |     warning('DC bus voltage must be positive.');
      |   end
      |   if (imax<=0)
      |     warning('Max. phase current must be positive.');
      |   end
      |   w0=6.283185307179586*wf0;
      |   pgain=2.0*wksi*w0*J/Kt;
      |   igain=w0*w0*J/Kt;
      |   fltPropGain=0.9*pgain;
      |   fltIntegGain=igain*SampleTime*0.5;
      |   if (Idmax<0)
      |     iratio=abs(Idmax)/imax;
      |     lowlim=acos(iratio)-1.570796326794897;
      |   else
      |     lowlim=0.0;
      |   end
      |   fltLowerLimit=lowlim;
      |   fltUpperLimit=0.0;
      |   fltLambda=lambdaFW;
      |   fltUmaxDivImax=0.5773502691896258*udcbus/imax;
      |   if isnan(fltUmaxDivImax)
      |     if ~strcmp(fltUmaxDivImax_bkup,'0')
      |       set_param(gcb,'fltUmaxDivImax','0');
      |     end
      |   else
      |     tmps=num2str(fltUmaxDivImax);
      |     if ~strcmp(fltUmaxDivImax_bkup,tmps)
      |       set_param(gcb,'fltUmaxDivImax',tmps);
      |     end
      |   end
      |   if isnan(fltLambda)
      |     if ~strcmp(fltLambda_bkup,'0')
      |       set_param(gcb,'fltLambda','0');
      |     end
      |   else
      |     tmps=num2str(fltLambda);
      |     if ~strcmp(fltLambda_bkup,tmps)
      |       set_param(gcb,'fltLambda',tmps);
      |     end
      |   end
      |   if isnan(fltPropGain)
      |     if ~strcmp(fltPropGain_bkup,'0')
      |       set_param(gcb,'fltPropGain','0');
      |     end
      |   else
      |     tmps=num2str(fltPropGain);
      |     if ~strcmp(fltPropGain_bkup,tmps)
      |       set_param(gcb,'fltPropGain',tmps);
      |     end
      |   end
      |   if isnan(fltIntegGain)
      |     if ~strcmp(fltIntegGain_bkup,'0')
      |       set_param(gcb,'fltIntegGain','0');
      |     end
      |   else
      |     tmps=num2str(fltIntegGain);
      |     if ~strcmp(fltIntegGain_bkup,tmps)
      |       set_param(gcb,'fltIntegGain',tmps);
      |     end
      |   end
      |   if isnan(fltLowerLimit)
      |     if ~strcmp(fltLowerLimit_bkup,'0')
      |       set_param(gcb,'fltLowerLimit','0');
      |     end
      |   else
      |     tmps=num2str(fltLowerLimit);
      |     if ~strcmp(fltLowerLimit_bkup,tmps)
      |       set_param(gcb,'fltLowerLimit',tmps);
      |     end
      |   end
      |   if isnan(fltUpperLimit)
      |     if ~strcmp(fltUpperLimit_bkup,'0')
      |       set_param(gcb,'fltUpperLimit','0');
      |     end
      |   else
      |     tmps=num2str(fltUpperLimit);
      |     if ~strcmp(fltUpperLimit_bkup,tmps)
      |       set_param(gcb,'fltUpperLimit',tmps);
      |     end
      |   end
      | end
      mask prompts: showStates "Show internal states:"; resetStatesEnable "Internal state after reset:"; showDebugOutputs "Show debugging outputs:"; SampleTime "Sample time (-1 for inherited):"; wf0 "Speed loop natural frequency f0 [Hz]:"; wksi "Speed loop attenuation ξ:"; J "Moment of inertia J [kg*m^2]:"; Kt "Motor torque constant Kt [N*m/A]:"; lambdaFW "Field weakening MA filter smoothing factor λ (0..1):"; Idmax "Maximum negative d-axis current (demagnetization current - CAUTION!) [A]:"; imax "Maximum phase current [A]:"; udcbus "DC bus voltage [V]:"; autoCalcEn "Calculate implementation parameters from physical parameters"; fltUmaxDivImax "fltUmaxDivImax (Maximal coil voltage divided by the maximal coil current):"; fltLambda "fltLambda (GDFLIB_FilterMA - smoothing factor):"; fltPropGain "fltPropGain (GFLIB_ControllerPIpAW - proportional gain):"; fltIntegGain "fltIntegGain (GFLIB_ControllerPIpAW - integral gain):"; fltLowerLimit "fltLowerLimit (GFLIB_ControllerPIpAW - lower limit):"; fltUpperLimit "fltUpperLimit (GFLIB_ControllerPIpAW - upper limit):"; SampleTime_1 "Discrete sample time:"
      mask help: Field Weakening controller for the PMSM field-oriented control algorithm in single precision floating-point implementation. This block supports re-initialization of the internal state during simulation. If the block is reset, the output of the MA filter and PI controller will be aligned with the inputs fltFilterMAFWOut_preset and fltControllerPIpAWFWOut_preset. Refer to the AMMCLIB User's Guide for further details.
      mask init:
      | ddName = get_param(bdroot,'DataDictionary');
      | if length(ddName)==0
      |   set_param(bdroot,'DataDictionary','ammclib_types.sldd');
      | else
      |   dd = Simulink.data.dictionary.open(ddName);
      |   data = getSection(dd,'Design Data');
      |   if ~exist(data,'SWLIBS_2Syst_F16')
      |     addDataSource(dd,'ammclib_types.sldd');
      |     saveChanges(dd);
      |   end
      | end
      | 
      | if showStates == 1
      |   % hidden state variables
      |   if strcmp(get_param([gcb '/fltUmaxDivImax'], 'BlockType'), 'Inport')
      |     posblk = get_param(gcb, 'Position');
      | 
      |     pos = get_param([gcb, '/fltUmaxDivImax'], 'Position');
      |     orient = get_param([gcb, '/fltUmaxDivImax'], 'Orientation');
      |     delete_block([gcb, '/fltUmaxDivImax']);
      |     add_block('built-in/Ground', [gcb, '/fltUmaxDivImax'], 'Position', pos, 'Orientation', orient);
      | 
      |     pos = get_param([gcb, '/fltLambda'], 'Position');
      |     orient = get_param([gcb, '/fltLambda'], 'Orientation');
      |     delete_block([gcb, '/fltLambda']);
      |     add_block('built-in/Ground', [gcb, '/fltLambda'], 'Position', pos, 'Orientation', orient);
      | 
      |     pos = get_param([gcb, '/fltPropGain'], 'Position');
      |     orient = get_param([gcb, '/fltPropGain'], 'Orientation');
      |     delete_block([gcb, '/fltPropGain']);
      |     add_block('built-in/Ground', [gcb, '/fltPropGain'], 'Position', pos, 'Orientation', orient);
      | 
      |     pos = get_param([gcb, '/fltIntegGain'], 'Position');
      |     orient = get_param([gcb, '/fltIntegGain'], 'Orientation');
      |     delete_block([gcb, '/fltIntegGain']);
      |     add_block('built-in/Ground', [gcb, '/fltIntegGain'], 'Position', pos, 'Orientation', orient);
      | 
      |     pos = get_param([gcb, '/fltLowerLimit'], 'Position');
      |     orient = get_param([gcb, '/fltLowerLimit'], 'Orientation');
      |     delete_block([gcb, '/fltLowerLimit']);
      |     add_block('built-in/Ground', [gcb, '/fltLowerLimit'], 'Position', pos, 'Orientation', orient);
      | 
      |     pos = get_param([gcb, '/fltUpperLimit'], 'Position');
      |     orient = get_param([gcb, '/fltUpperLimit'], 'Orientation');
      |     delete_block([gcb, '/fltUpperLimit']);
      |     add_block('built-in/Ground', [gcb, '/fltUpperLimit'], 'Position', pos, 'Orientation', orient);
      | 
      |     pos = get_param([gcb, '/fltIQReqK_1'], 'Position');
      |     orient = get_param([gcb, '/fltIQReqK_1'], 'Orientation');
      |     delete_block([gcb, '/fltIQReqK_1']);
      |     add_block('built-in/Ground', [gcb, '/fltIQReqK_1'], 'Position', pos, 'Orientation', orient);
      | 
      |     pos = get_param([gcb, '/fltAcc'], 'Position');
      |     orient = get_param([gcb, '/fltAcc'], 'Orientation');
      |     delete_block([gcb, '/fltAcc']);
      |     add_block('built-in/Ground', [gcb, '/fltAcc'], 'Position', pos, 'Orientation', orient);
      | 
      |     pos = get_param([gcb, '/fltIntegPartK_1'], 'Position');
      |     orient = get_param([gcb, '/fltIntegPartK_1'], 'Orientation');
      |     delete_block([gcb, '/fltIntegPartK_1']);
      |     add_block('built-in/Ground', [gcb, '/fltIntegPartK_1'], 'Position', pos, 'Orientation', orient);
      | 
      |     pos = get_param([gcb, '/fltInK_1'], 'Position');
      |     orient = get_param([gcb, '/fltInK_1'], 'Orientation');
      |     delete_block([gcb, '/fltInK_1']);
      |     add_block('built-in/Ground', [gcb, '/fltInK_1'], 'Position', pos, 'Orientation', orient);
      | 
      | 
      |     pmask=Simulink.Mask.get(gcb);
      |     pctrl=pmask.getParameter('SampleTime');
      |     pctrl.set('TypeOptions',{'fltIDQReqAmp/SampleTime','fltVelocityFbck/SampleTime','fltIQFbck/SampleTime','fltUQReq/SampleTime','fltUQLim/SampleTime','fltFilterMAFWOut_preset/SampleTime','fltControllerPIpAWFWOut_preset/SampleTime'});
      | 
      |     pos = get_param([gcb '/fltAcc_Out'], 'Position');
      |     orient = get_param([gcb '/fltAcc_Out'], 'Orientation');
      |     delete_block([gcb '/fltAcc_Out']);
      |     add_block('built-in/Terminator', [gcb '/fltAcc_Out'], 'Position', pos, 'Orientation', orient);
      | 
      |     pos = get_param([gcb '/fltIntegPartK_1_Out'], 'Position');
      |     orient = get_param([gcb '/fltIntegPartK_1_Out'], 'Orientation');
      |     delete_block([gcb '/fltIntegPartK_1_Out']);
      |     add_block('built-in/Terminator', [gcb '/fltIntegPartK_1_Out'], 'Position', pos, 'Orientation', orient);
      | 
      |     pos = get_param([gcb '/fltInK_1_Out'], 'Position');
      |     orient = get_param([gcb '/fltInK_1_Out'], 'Orientation');
      |     delete_block([gcb '/fltInK_1_Out']);
      |     add_block('built-in/Terminator', [gcb '/fltInK_1_Out'], 'Position', pos, 'Orientation', orient);
      | 
      |     if strcmp(get_param([gcb '/fltIQErrSign'], 'BlockType'), 'Outport')
      |       pos = get_param([gcb '/fltIQErrSign'], 'Position');
      |       orient = get_param([gcb '/fltIQErrSign'], 'Orientation');
      |       delete_block([gcb '/fltIQErrSign']);
      |       add_block('built-in/Terminator', [gcb '/fltIQErrSign'], 'Position', pos, 'Orientation', orient);
      | 
      |       pos = get_param([gcb '/fltIQErr'], 'Position');
      |       orient = get_param([gcb '/fltIQErr'], 'Orientation');
      |       delete_block([gcb '/fltIQErr']);
      |       add_block('built-in/Terminator', [gcb '/fltIQErr'], 'Position', pos, 'Orientation', orient);
      | 
      |       pos = get_param([gcb '/fltFWErr'], 'Position');
      |       orient = get_param([gcb '/fltFWErr'], 'Orientation');
      |       delete_block([gcb '/fltFWErr']);
      |       add_block('built-in/Terminator', [gcb '/fltFWErr'], 'Position', pos, 'Orientation', orient);
      | 
      |       pos = get_param([gcb '/fltUQErr'], 'Position');
      |       orient = get_param([gcb '/fltUQErr'], 'Orientation');
      |       delete_block([gcb '/fltUQErr']);
      |       add_block('built-in/Terminator', [gcb '/fltUQErr'], 'Position', pos, 'Orientation', orient);
      | 
      |       pos = get_param([gcb '/fltFWErrFilt'], 'Position');
      |       orient = get_param([gcb '/fltFWErrFilt'], 'Orientation');
      |       delete_block([gcb '/fltFWErrFilt']);
      |       add_block('built-in/Terminator', [gcb '/fltFWErrFilt'], 'Position', pos, 'Orientation', orient);
      | 
      |       pos = get_param([gcb '/fltFWAngle'], 'Position');
      |       orient = get_param([gcb '/fltFWAngle'], 'Orientation');
      |       delete_block([gcb '/fltFWAngle']);
      |       add_block('built-in/Terminator', [gcb '/fltFWAngle'], 'Position', pos, 'Orientation', orient);
      | 
      |       pos = get_param([gcb '/fltFWSin'], 'Position');
      |       orient = get_param([gcb '/fltFWSin'], 'Orientation');
      |       delete_block([gcb '/fltFWSin']);
      |       add_block('built-in/Terminator', [gcb '/fltFWSin'], 'Position', pos, 'Orientation', orient);
      | 
      |       pos = get_param([gcb '/fltFWCos'], 'Position');
      |       orient = get_param([gcb '/fltFWCos'], 'Orientation');
      |       delete_block([gcb '/fltFWCos']);
      |       add_block('built-in/Terminator', [gcb '/fltFWCos'], 'Position', pos, 'Orientation', orient);
      | 
      |     end
      | 
      |     set_param([gcb '/fltIDQReqAmp'], 'Port', '1');
      |     set_param([gcb '/fltVelocityFbck'], 'Port', '2');
      |     set_param([gcb '/fltIQFbck'], 'Port', '3');
      |     set_param([gcb '/fltUQReq'], 'Port', '4');
      |     set_param([gcb '/fltUQLim'], 'Port', '5');
      |     set_param([gcb '/fltFilterMAFWOut_preset'], 'Port', '6');
      |     set_param([gcb '/fltControllerPIpAWFWOut_preset'], 'Port', '7');
      | 
      |     tmpOutCnt=0;
      |     tmpOutCnt=tmpOutCnt+1;
      |     set_param([gcb '/pIDQReq'], 'Port', num2str(tmpOutCnt));
      |     tmpOutCnt=tmpOutCnt+1;
      |     set_param([gcb '/u16LimitFlag'], 'Port', num2str(tmpOutCnt));
      | 
      |     autoCalcEn=get_param(gcb,'autoCalcEn');
      |     if strcmp(autoCalcEn,'on')
      |       set_param(gcb,'MaskEnables',{'on','on','off','on','on','on','on','on','on','on','on','on','on','on','on','on','on','on','on','off'});
      |     else
      |       set_param(gcb,'MaskEnables',{'on','on','off','on','off','off','off','off','off','off','off','off','on','on','on','on','on','on','on','off'});
      |     end
      | 
      |     if (posblk(4) - posblk(2)) > 200
      |       height = 200;
      |       set_param(gcb,'Position',[posblk(1), posblk(2), posblk(3), posblk(2)+height])
      |     end
      |   end
      | else
      |   % shown state variables
      |   if strcmp(get_param([gcb '/fltUmaxDivImax'], 'BlockType'), 'Ground')
      |     posblk = get_param(gcb, 'Position');
      | 
      |     pos = get_param([gcb, '/fltUmaxDivImax'], 'Position');
      |     orient = get_param([gcb, '/fltUmaxDivImax'], 'Orientation');
      |     delete_block([gcb, '/fltUmaxDivImax']);
      |     add_block('built-in/Inport', [gcb, '/fltUmaxDivImax'], 'Position', pos, 'Orientation', orient, 'OutDataTypeStr', 'single');
      | 
      |     pos = get_param([gcb, '/fltLambda'], 'Position');
      |     orient = get_param([gcb, '/fltLambda'], 'Orientation');
      |     delete_block([gcb, '/fltLambda']);
      |     add_block('built-in/Inport', [gcb, '/fltLambda'], 'Position', pos, 'Orientation', orient, 'OutDataTypeStr', 'single');
      | 
      |     pos = get_param([gcb, '/fltPropGain'], 'Position');
      |     orient = get_param([gcb, '/fltPropGain'], 'Orientation');
      |     delete_block([gcb, '/fltPropGain']);
      |     add_block('built-in/Inport', [gcb, '/fltPropGain'], 'Position', pos, 'Orientation', orient, 'OutDataTypeStr', 'single');
      | 
      |     pos = get_param([gcb, '/fltIntegGain'], 'Position');
      |     orient = get_param([gcb, '/fltIntegGain'], 'Orientation');
      |     delete_block([gcb, '/fltIntegGain']);
      |     add_block('built-in/Inport', [gcb, '/fltIntegGain'], 'Position', pos, 'Orientation', orient, 'OutDataTypeStr', 'single');
      | 
      |     pos = get_param([gcb, '/fltLowerLimit'], 'Position');
      |     orient = get_param([gcb, '/fltLowerLimit'], 'Orientation');
      |     delete_block([gcb, '/fltLowerLimit']);
      |     add_block('built-in/Inport', [gcb, '/fltLowerLimit'], 'Position', pos, 'Orientation', orient, 'OutDataTypeStr', 'single');
      | 
      |     pos = get_param([gcb, '/fltUpperLimit'], 'Position');
      |     orient = get_param([gcb, '/fltUpperLimit'], 'Orientation');
      |     delete_block([gcb, '/fltUpperLimit']);
      |     add_block('built-in/Inport', [gcb, '/fltUpperLimit'], 'Position', pos, 'Orientation', orient, 'OutDataTypeStr', 'single');
      | 
      |     pos = get_param([gcb, '/fltIQReqK_1'], 'Position');
      |     orient = get_param([gcb, '/fltIQReqK_1'], 'Orientation');
      |     delete_block([gcb, '/fltIQReqK_1']);
      |     add_block('built-in/Inport', [gcb, '/fltIQReqK_1'], 'Position', pos, 'Orientation', orient, 'OutDataTypeStr', 'single');
      | 
      |     pos = get_param([gcb, '/fltAcc'], 'Position');
      |     orient = get_param([gcb, '/fltAcc'], 'Orientation');
      |     delete_block([gcb, '/fltAcc']);
      |     add_block('built-in/Inport', [gcb, '/fltAcc'], 'Position', pos, 'Orientation', orient, 'OutDataTypeStr', 'single');
      | 
      |     pos = get_param([gcb, '/fltIntegPartK_1'], 'Position');
      |     orient = get_param([gcb, '/fltIntegPartK_1'], 'Orientation');
      |     delete_block([gcb, '/fltIntegPartK_1']);
      |     add_block('built-in/Inport', [gcb, '/fltIntegPartK_1'], 'Position', pos, 'Orientation', orient, 'OutDataTypeStr', 'single');
      | 
      |     pos = get_param([gcb, '/fltInK_1'], 'Position');
      |     orient = get_param([gcb, '/fltInK_1'], 'Orientation');
      |     delete_block([gcb, '/fltInK_1']);
      |     add_block('built-in/Inport', [gcb, '/fltInK_1'], 'Position', pos, 'Orientation', orient, 'OutDataTypeStr', 'single');
      | 
      | 
      | 
      |     pos = get_param([gcb '/fltAcc_Out'], 'Position');
      |     orient = get_param([gcb '/fltAcc_Out'], 'Orientation');
      |     delete_block([gcb '/fltAcc_Out']);
      |     add_block('built-in/Outport', [gcb '/fltAcc_Out'], 'Position', pos, 'Orientation', orient);
      | 
      |     pos = get_param([gcb '/fltIntegPartK_1_Out'], 'Position');
      |     orient = get_param([gcb '/fltIntegPartK_1_Out'], 'Orientation');
      |     delete_block([gcb '/fltIntegPartK_1_Out']);
      |     add_block('built-in/Outport', [gcb '/fltIntegPartK_1_Out'], 'Position', pos, 'Orientation', orient);
      | 
      |     pos = get_param([gcb '/fltInK_1_Out'], 'Position');
      |     orient = get_param([gcb '/fltInK_1_Out'], 'Orientation');
      |     delete_block([gcb '/fltInK_1_Out']);
      |     add_block('built-in/Outport', [gcb '/fltInK_1_Out'], 'Position', pos, 'Orientation', orient);
      | 
      | 
      |     pmask=Simulink.Mask.get(gcb);
      |     pctrl=pmask.getParameter('SampleTime');
      |     pctrl.set('TypeOptions',{'fltIDQReqAmp/SampleTime','fltVelocityFbck/SampleTime','fltIQFbck/SampleTime','fltUQReq/SampleTime','fltUQLim/SampleTime','fltFilterMAFWOut_preset/SampleTime','fltControllerPIpAWFWOut_preset/SampleTime','fltUmaxDivImax/SampleTime','fltLambda/SampleTime','fltPropGain/SampleTime','fltIntegGain/SampleTime','fltLowerLimit/SampleTime','fltUpperLimit/SampleTime','fltIQReqK_1/SampleTime','fltAcc/SampleTime','fltIntegPartK_1/SampleTime','fltInK_1/SampleTime'});
      | 
      |     if (showDebugOutputs == 2) && (strcmp(get_param([gcb '/fltIQErrSign'], 'BlockType'), 'Terminator'))
      |       pos = get_param([gcb '/fltIQErrSign'], 'Position');
      |       orient = get_param([gcb '/fltIQErrSign'], 'Orientation');
      |       delete_block([gcb '/fltIQErrSign']);
      |       add_block('built-in/Outport', [gcb '/fltIQErrSign'], 'Position', pos, 'Orientation', orient);
      | 
      |       pos = get_param([gcb '/fltIQErr'], 'Position');
      |       orient = get_param([gcb '/fltIQErr'], 'Orientation');
      |       delete_block([gcb '/fltIQErr']);
      |       add_block('built-in/Outport', [gcb '/fltIQErr'], 'Position', pos, 'Orientation', orient);
      | 
      |       pos = get_param([gcb '/fltFWErr'], 'Position');
      |       orient = get_param([gcb '/fltFWErr'], 'Orientation');
      |       delete_block([gcb '/fltFWErr']);
      |       add_block('built-in/Outport', [gcb '/fltFWErr'], 'Position', pos, 'Orientation', orient);
      | 
      |       pos = get_param([gcb '/fltUQErr'], 'Position');
      |       orient = get_param([gcb '/fltUQErr'], 'Orientation');
      |       delete_block([gcb '/fltUQErr']);
      |       add_block('built-in/Outport', [gcb '/fltUQErr'], 'Position', pos, 'Orientation', orient);
      | 
      |       pos = get_param([gcb '/fltFWErrFilt'], 'Position');
      |       orient = get_param([gcb '/fltFWErrFilt'], 'Orientation');
      |       delete_block([gcb '/fltFWErrFilt']);
      |       add_block('built-in/Outport', [gcb '/fltFWErrFilt'], 'Position', pos, 'Orientation', orient);
      | 
      |       pos = get_param([gcb '/fltFWAngle'], 'Position');
      |       orient = get_param([gcb '/fltFWAngle'], 'Orientation');
      |       delete_block([gcb '/fltFWAngle']);
      |       add_block('built-in/Outport', [gcb '/fltFWAngle'], 'Position', pos, 'Orientation', orient);
      | 
      |       pos = get_param([gcb '/fltFWSin'], 'Position');
      |       orient = get_param([gcb '/fltFWSin'], 'Orientation');
      |       delete_block([gcb '/fltFWSin']);
      |       add_block('built-in/Outport', [gcb '/fltFWSin'], 'Position', pos, 'Orientation', orient);
      | 
      |       pos = get_param([gcb '/fltFWCos'], 'Position');
      |       orient = get_param([gcb '/fltFWCos'], 'Orientation');
      |       delete_block([gcb '/fltFWCos']);
      |       add_block('built-in/Outport', [gcb '/fltFWCos'], 'Position', pos, 'Orientation', orient);
      | 
      |     end
      | 
      |     set_param([gcb '/fltIDQReqAmp'], 'Port', '1');
      |     set_param([gcb '/fltVelocityFbck'], 'Port', '2');
      |     set_param([gcb '/fltIQFbck'], 'Port', '3');
      |     set_param([gcb '/fltUQReq'], 'Port', '4');
      |     set_param([gcb '/fltUQLim'], 'Port', '5');
      |     set_param([gcb '/fltFilterMAFWOut_preset'], 'Port', '6');
      |     set_param([gcb '/fltControllerPIpAWFWOut_preset'], 'Port', '7');
      |     set_param([gcb '/fltUmaxDivImax'], 'Port', '8');
      |     set_param([gcb '/fltLambda'], 'Port', '9');
      |     set_param([gcb '/fltPropGain'], 'Port', '10');
      |     set_param([gcb '/fltIntegGain'], 'Port', '11');
      |     set_param([gcb '/fltLowerLimit'], 'Port', '12');
      |     set_param([gcb '/fltUpperLimit'], 'Port', '13');
      |     set_param([gcb '/fltIQReqK_1'], 'Port', '14');
      |     set_param([gcb '/fltAcc'], 'Port', '15');
      |     set_param([gcb '/fltIntegPartK_1'], 'Port', '16');
      |     set_param([gcb '/fltInK_1'], 'Port', '17');
      | 
      |     if (showDebugOutputs == 2)
      |       tmpOutCnt=0;
      |       tmpOutCnt=tmpOutCnt+1;
      |       set_param([gcb '/pIDQReq'], 'Port', num2str(tmpOutCnt));
      |       tmpOutCnt=tmpOutCnt+1;
      |       set_param([gcb '/u16LimitFlag'], 'Port', num2str(tmpOutCnt));
      |       tmpOutCnt=tmpOutCnt+1;
      |       set_param([gcb '/fltIQErrSign'], 'Port', num2str(tmpOutCnt));
      |       tmpOutCnt=tmpOutCnt+1;
      |       set_param([gcb '/fltIQErr'], 'Port', num2str(tmpOutCnt));
      |       tmpOutCnt=tmpOutCnt+1;
      |       set_param([gcb '/fltFWErr'], 'Port', num2str(tmpOutCnt));
      |       tmpOutCnt=tmpOutCnt+1;
      |       set_param([gcb '/fltUQErr'], 'Port', num2str(tmpOutCnt));
      |       tmpOutCnt=tmpOutCnt+1;
      |       set_param([gcb '/fltFWErrFilt'], 'Port', num2str(tmpOutCnt));
      |       tmpOutCnt=tmpOutCnt+1;
      |       set_param([gcb '/fltFWAngle'], 'Port', num2str(tmpOutCnt));
      |       tmpOutCnt=tmpOutCnt+1;
      |       set_param([gcb '/fltFWSin'], 'Port', num2str(tmpOutCnt));
      |       tmpOutCnt=tmpOutCnt+1;
      |       set_param([gcb '/fltFWCos'], 'Port', num2str(tmpOutCnt));
      |       tmpOutCnt=tmpOutCnt+1;
      |       set_param([gcb '/fltAcc_Out'], 'Port', num2str(tmpOutCnt));
      |       tmpOutCnt=tmpOutCnt+1;
      |       set_param([gcb '/fltIntegPartK_1_Out'], 'Port', num2str(tmpOutCnt));
      |       tmpOutCnt=tmpOutCnt+1;
      |       set_param([gcb '/fltInK_1_Out'], 'Port', num2str(tmpOutCnt));
      |     else
      |       tmpOutCnt=0;
      |       tmpOutCnt=tmpOutCnt+1;
      |       set_param([gcb '/pIDQReq'], 'Port', num2str(tmpOutCnt));
      |       tmpOutCnt=tmpOutCnt+1;
      |       set_param([gcb '/u16LimitFlag'], 'Port', num2str(tmpOutCnt));
      |       tmpOutCnt=tmpOutCnt+1;
      |       set_param([gcb '/fltAcc_Out'], 'Port', num2str(tmpOutCnt));
      |       tmpOutCnt=tmpOutCnt+1;
      |       set_param([gcb '/fltIntegPartK_1_Out'], 'Port', num2str(tmpOutCnt));
      |       tmpOutCnt=tmpOutCnt+1;
      |       set_param([gcb '/fltInK_1_Out'], 'Port', num2str(tmpOutCnt));
      |     end
      | 
      |     set_param(gcb,'MaskEnables',{'on','on','on','on','off','off','off','off','off','off','off','off','off','off','off','off','off','off','off','off'});
      | 
      |     if (posblk(4) - posblk(2)) < 450
      |       height = 450;
      |       set_param(gcb,'Position',[posblk(1), posblk(2), posblk(3), posblk(2)+height])
      |     end
      |   else
      |     if (showDebugOutputs == 2) && (strcmp(get_param([gcb '/fltIQErrSign'], 'BlockType'), 'Terminator'))
      |       % shown debugging outputs
      |       pos = get_param([gcb '/fltIQErrSign'], 'Position');
      |       orient = get_param([gcb '/fltIQErrSign'], 'Orientation');
      |       delete_block([gcb '/fltIQErrSign']);
      |       add_block('built-in/Outport', [gcb '/fltIQErrSign'], 'Position', pos, 'Orientation', orient);
      | 
      |       pos = get_param([gcb '/fltIQErr'], 'Position');
      |       orient = get_param([gcb '/fltIQErr'], 'Orientation');
      |       delete_block([gcb '/fltIQErr']);
      |       add_block('built-in/Outport', [gcb '/fltIQErr'], 'Position', pos, 'Orientation', orient);
      | 
      |       pos = get_param([gcb '/fltFWErr'], 'Position');
      |       orient = get_param([gcb '/fltFWErr'], 'Orientation');
      |       delete_block([gcb '/fltFWErr']);
      |       add_block('built-in/Outport', [gcb '/fltFWErr'], 'Position', pos, 'Orientation', orient);
      | 
      |       pos = get_param([gcb '/fltUQErr'], 'Position');
      |       orient = get_param([gcb '/fltUQErr'], 'Orientation');
      |       delete_block([gcb '/fltUQErr']);
      |       add_block('built-in/Outport', [gcb '/fltUQErr'], 'Position', pos, 'Orientation', orient);
      | 
      |       pos = get_param([gcb '/fltFWErrFilt'], 'Position');
      |       orient = get_param([gcb '/fltFWErrFilt'], 'Orientation');
      |       delete_block([gcb '/fltFWErrFilt']);
      |       add_block('built-in/Outport', [gcb '/fltFWErrFilt'], 'Position', pos, 'Orientation', orient);
      | 
      |       pos = get_param([gcb '/fltFWAngle'], 'Position');
      |       orient = get_param([gcb '/fltFWAngle'], 'Orientation');
      |       delete_block([gcb '/fltFWAngle']);
      |       add_block('built-in/Outport', [gcb '/fltFWAngle'], 'Position', pos, 'Orientation', orient);
      | 
      |       pos = get_param([gcb '/fltFWSin'], 'Position');
      |       orient = get_param([gcb '/fltFWSin'], 'Orientation');
      |       delete_block([gcb '/fltFWSin']);
      |       add_block('built-in/Outport', [gcb '/fltFWSin'], 'Position', pos, 'Orientation', orient);
      | 
      |       pos = get_param([gcb '/fltFWCos'], 'Position');
      |       orient = get_param([gcb '/fltFWCos'], 'Orientation');
      |       delete_block([gcb '/fltFWCos']);
      |       add_block('built-in/Outport', [gcb '/fltFWCos'], 'Position', pos, 'Orientation', orient);
      | 
      |       tmpOutCnt=0;
      |       tmpOutCnt=tmpOutCnt+1;
      |       set_param([gcb '/pIDQReq'], 'Port', num2str(tmpOutCnt));
      |       tmpOutCnt=tmpOutCnt+1;
      |       set_param([gcb '/u16LimitFlag'], 'Port', num2str(tmpOutCnt));
      |       tmpOutCnt=tmpOutCnt+1;
      |       set_param([gcb '/fltIQErrSign'], 'Port', num2str(tmpOutCnt));
      |       tmpOutCnt=tmpOutCnt+1;
      |       set_param([gcb '/fltIQErr'], 'Port', num2str(tmpOutCnt));
      |       tmpOutCnt=tmpOutCnt+1;
      |       set_param([gcb '/fltFWErr'], 'Port', num2str(tmpOutCnt));
      |       tmpOutCnt=tmpOutCnt+1;
      |       set_param([gcb '/fltUQErr'], 'Port', num2str(tmpOutCnt));
      |       tmpOutCnt=tmpOutCnt+1;
      |       set_param([gcb '/fltFWErrFilt'], 'Port', num2str(tmpOutCnt));
      |       tmpOutCnt=tmpOutCnt+1;
      |       set_param([gcb '/fltFWAngle'], 'Port', num2str(tmpOutCnt));
      |       tmpOutCnt=tmpOutCnt+1;
      |       set_param([gcb '/fltFWSin'], 'Port', num2str(tmpOutCnt));
      |       tmpOutCnt=tmpOutCnt+1;
      |       set_param([gcb '/fltFWCos'], 'Port', num2str(tmpOutCnt));
      |       tmpOutCnt=tmpOutCnt+1;
      |       set_param([gcb '/fltAcc_Out'], 'Port', num2str(tmpOutCnt));
      |       tmpOutCnt=tmpOutCnt+1;
      |       set_param([gcb '/fltIntegPartK_1_Out'], 'Port', num2str(tmpOutCnt));
      |       tmpOutCnt=tmpOutCnt+1;
      |       set_param([gcb '/fltInK_1_Out'], 'Port', num2str(tmpOutCnt));
      |     elseif (showDebugOutputs == 1) && (strcmp(get_param([gcb '/fltIQErrSign'], 'BlockType'), 'Outport'))
      |       % hidden debugging outputs
      |       pos = get_param([gcb '/fltIQErrSign'], 'Position');
      |       orient = get_param([gcb '/fltIQErrSign'], 'Orientation');
      |       delete_block([gcb '/fltIQErrSign']);
      |       add_block('built-in/Terminator', [gcb '/fltIQErrSign'], 'Position', pos, 'Orientation', orient);
      | 
      |       pos = get_param([gcb '/fltIQErr'], 'Position');
      |       orient = get_param([gcb '/fltIQErr'], 'Orientation');
      |       delete_block([gcb '/fltIQErr']);
      |       add_block('built-in/Terminator', [gcb '/fltIQErr'], 'Position', pos, 'Orientation', orient);
      | 
      |       pos = get_param([gcb '/fltFWErr'], 'Position');
      |       orient = get_param([gcb '/fltFWErr'], 'Orientation');
      |       delete_block([gcb '/fltFWErr']);
      |       add_block('built-in/Terminator', [gcb '/fltFWErr'], 'Position', pos, 'Orientation', orient);
      | 
      |       pos = get_param([gcb '/fltUQErr'], 'Position');
      |       orient = get_param([gcb '/fltUQErr'], 'Orientation');
      |       delete_block([gcb '/fltUQErr']);
      |       add_block('built-in/Terminator', [gcb '/fltUQErr'], 'Position', pos, 'Orientation', orient);
      | 
      |       pos = get_param([gcb '/fltFWErrFilt'], 'Position');
      |       orient = get_param([gcb '/fltFWErrFilt'], 'Orientation');
      |       delete_block([gcb '/fltFWErrFilt']);
      |       add_block('built-in/Terminator', [gcb '/fltFWErrFilt'], 'Position', pos, 'Orientation', orient);
      | 
      |       pos = get_param([gcb '/fltFWAngle'], 'Position');
      |       orient = get_param([gcb '/fltFWAngle'], 'Orientation');
      |       delete_block([gcb '/fltFWAngle']);
      |       add_block('built-in/Terminator', [gcb '/fltFWAngle'], 'Position', pos, 'Orientation', orient);
      | 
      |       pos = get_param([gcb '/fltFWSin'], 'Position');
      |       orient = get_param([gcb '/fltFWSin'], 'Orientation');
      |       delete_block([gcb '/fltFWSin']);
      |       add_block('built-in/Terminator', [gcb '/fltFWSin'], 'Position', pos, 'Orientation', orient);
      | 
      |       pos = get_param([gcb '/fltFWCos'], 'Position');
      |       orient = get_param([gcb '/fltFWCos'], 'Orientation');
      |       delete_block([gcb '/fltFWCos']);
      |       add_block('built-in/Terminator', [gcb '/fltFWCos'], 'Position', pos, 'Orientation', orient);
      | 
      |       tmpOutCnt=0;
      |       tmpOutCnt=tmpOutCnt+1;
      |       set_param([gcb '/pIDQReq'], 'Port', num2str(tmpOutCnt));
      |       tmpOutCnt=tmpOutCnt+1;
      |       set_param([gcb '/u16LimitFlag'], 'Port', num2str(tmpOutCnt));
      |       tmpOutCnt=tmpOutCnt+1;
      |       set_param([gcb '/fltAcc_Out'], 'Port', num2str(tmpOutCnt));
      |       tmpOutCnt=tmpOutCnt+1;
      |       set_param([gcb '/fltIntegPartK_1_Out'], 'Port', num2str(tmpOutCnt));
      |       tmpOutCnt=tmpOutCnt+1;
      |       set_param([gcb '/fltInK_1_Out'], 'Port', num2str(tmpOutCnt));
      |     end
      |   end
      | end
      settings: RTWSystemCode=Inline
      mask Help: web([fileparts(which('ammclib_bam_S32K3xx.slx')) '/../doc/S32K3XXMCLUG.pdf'], '-browser')
      mask TypeOptions showStates: Hide (faster execution) | Show (allows debugging; connect feedback loops manually)
      mask Callback showStates:
      | maskStr=get_param(gcb,'showStates');
      | if strcmp(maskStr,'Hide (faster execution)')
      |   if strcmp(get_param([gcb '/fltUmaxDivImax'], 'BlockType'), 'Inport')
      |     autoCalcEn=get_param(gcb,'autoCalcEn');
      |     if strcmp(autoCalcEn,'on')
      |       set_param(gcb,'MaskEnables',{'on','on','off','on','on','on','on','on','on','on','on','on','on','on','on','on','on','on','on','off'});
      |     else
      |       set_param(gcb,'MaskEnables',{'on','on','off','on','off','off','off','off','off','off','off','off','on','on','on','on','on','on','on','off'});
      |     end
      |   end
      | else
      |   if strcmp(get_param([gcb '/fltUmaxDivImax'], 'BlockType'), 'Ground')
      |     set_param(gcb,'MaskEnables',{'on','on','on','on','off','off','off','off','off','off','off','off','off','off','off','off','off','off','off','off'});
      |   end
      | end
      mask TypeOptions resetStatesEnable: Pre-set according to the first set of inputs after reset | Clear to zero
      mask TypeOptions showDebugOutputs: Hide | Show
      mask TypeOptions SampleTime: fltIDQReqAmp/SampleTime | fltVelocityFbck/SampleTime | fltIQFbck/SampleTime | fltUQReq/SampleTime | fltUQLim/SampleTime | fltFilterMAFWOut_preset/SampleTime | fltControllerPIpAWFWOut_preset/SampleTime
      mask Callback SampleTime:
      | p=Simulink.Mask.get(gcb);
      | hintText=p.getDialogControl('timeHint');
      | SampleTime=Simulink.data.evalinGlobal(bdroot,get_param(gcb,'SampleTime'));
      | SampleTime_1=str2double(get_param(gcb,'SampleTime_1'));
      | if (((SampleTime==-1) && (~contains(hintText.Prompt,'inherited'))) || ...
      |     ((SampleTime~=-1) && contains(hintText.Prompt,'inherited')) || ...
      |     ((SampleTime~=-1) && (SampleTime_1~=SampleTime)) || ...
      |     ((SampleTime_1~=-1) && contains(hintText.Prompt,'yet')))
      |   if ((SampleTime==-1) && (~contains(hintText.Prompt,'inherited')))
      |     set_param(gcb,'SampleTime_1',num2str(NaN));
      |     SampleTime_1=NaN;
      |   end
      |   if (SampleTime~=-1)
      |     set_param(gcb,'SampleTime_1',num2str(SampleTime));
      |     SampleTime_1=SampleTime;
      |   end
      |   autoCalcEn=get_param(gcb,'autoCalcEn');
      |   if strcmp(autoCalcEn,'on')
      |     p=Simulink.Mask.get(gcb);
      |     hintText=p.getDialogControl('timeHint');
      |     if SampleTime==-1
      |       SampleTime=SampleTime_1;
      |       if isnan(SampleTime)
      |         hintText.Prompt='Note: Implementation parameters cannot be calculated yet because the block''s inherited sample time is unknown. Simulink will update the sample time when you run the simulation.';
      |       else
      |         hintText.Prompt='Caution: Implementation parameters depend on inherited sample time. Make sure that the sample time of the block''s inputs corresponds to the sampling period in the target application.';
      |       end
      |     else
      |       hintText.Prompt='Caution: Implementation parameters depend on the sample time. Make sure that the simulation time step corresponds to the sampling period in the target application.';
      |     end
      |     fltUmaxDivImax_bkup=get_param(gcb,'fltUmaxDivImax');
      |     fltLambda_bkup=get_param(gcb,'fltLambda');
      |     fltPropGain_bkup=get_param(gcb,'fltPropGain');
      |     fltIntegGain_bkup=get_param(gcb,'fltIntegGain');
      |     fltLowerLimit_bkup=get_param(gcb,'fltLowerLimit');
      |     fltUpperLimit_bkup=get_param(gcb,'fltUpperLimit');
      |     wf0=Simulink.data.evalinGlobal(bdroot,get_param(gcb,'wf0'));
      |     wksi=Simulink.data.evalinGlobal(bdroot,get_param(gcb,'wksi'));
      |     J=Simulink.data.evalinGlobal(bdroot,get_param(gcb,'J'));
      |     Kt=Simulink.data.evalinGlobal(bdroot,get_param(gcb,'Kt'));
      |     lambdaFW=Simulink.data.evalinGlobal(bdroot,get_param(gcb,'lambdaFW'));
      |     Idmax=Simulink.data.evalinGlobal(bdroot,get_param(gcb,'Idmax'));
      |     imax=Simulink.data.evalinGlobal(bdroot,get_param(gcb,'imax'));
      |     udcbus=Simulink.data.evalinGlobal(bdroot,get_param(gcb,'udcbus'));
      |     if (wf0<=0)
      |       warning('Natural frequency f0 must be positive.');
      |     end
      |     if (wksi<=0)
      |       warning('Current loop attenuation must be positive.');
      |     end
      |     if (wksi>1)
      |       warning('Current loop attenuation must not exceed 1.');
      |     end
      |     if (J<=0)
      |       warning('Moment of inertia J must be positive.');
      |     end
      |     if (Kt<=0)
      |       warning('Torque constant Kt must be positive.');
      |     end
      |     if (lambdaFW<0)
      |       warning('MA filter smoothing factor must be in the range 0..1.');
      |     end
      |     if (lambdaFW>1)
      |       warning('MA filter smoothing factor must be in the range 0..1.');
      |     end
      |     if (udcbus<=0)
      |       warning('DC bus voltage must be positive.');
      |     end
      |     if (imax<=0)
      |       warning('Max. phase current must be positive.');
      |     end
      |     w0=6.283185307179586*wf0;
      |     pgain=2.0*wksi*w0*J/Kt;
      |     igain=w0*w0*J/Kt;
      |     fltPropGain=0.9*pgain;
      |     fltIntegGain=igain*SampleTime*0.5;
      |     if (Idmax<0)
      |       iratio=abs(Idmax)/imax;
      |       lowlim=acos(iratio)-1.570796326794897;
      |     else
      |       lowlim=0.0;
      |     end
      |     fltLowerLimit=lowlim;
      |     fltUpperLimit=0.0;
      |     fltLambda=lambdaFW;
      |     fltUmaxDivImax=0.5773502691896258*udcbus/imax;
      |     if isnan(fltUmaxDivImax)
      |       if ~strcmp(fltUmaxDivImax_bkup,'0')
      |         set_param(gcb,'fltUmaxDivImax','0');
      |       end
      |     else
      |       tmps=num2str(fltUmaxDivImax);
      |       if ~strcmp(fltUmaxDivImax_bkup,tmps)
      |         set_param(gcb,'fltUmaxDivImax',tmps);
      |       end
      |     end
      |     if isnan(fltLambda)
      |       if ~strcmp(fltLambda_bkup,'0')
      |         set_param(gcb,'fltLambda','0');
      |       end
      |     else
      |       tmps=num2str(fltLambda);
      |       if ~strcmp(fltLambda_bkup,tmps)
      |         set_param(gcb,'fltLambda',tmps);
      |       end
      |     end
      |     if isnan(fltPropGain)
      |       if ~strcmp(fltPropGain_bkup,'0')
      |         set_param(gcb,'fltPropGain','0');
      |       end
      |     else
      |       tmps=num2str(fltPropGain);
      |       if ~strcmp(fltPropGain_bkup,tmps)
      |         set_param(gcb,'fltPropGain',tmps);
      |       end
      |     end
      |     if isnan(fltIntegGain)
      |       if ~strcmp(fltIntegGain_bkup,'0')
      |         set_param(gcb,'fltIntegGain','0');
      |       end
      |     else
      |       tmps=num2str(fltIntegGain);
      |       if ~strcmp(fltIntegGain_bkup,tmps)
      |         set_param(gcb,'fltIntegGain',tmps);
      |       end
      |     end
      |     if isnan(fltLowerLimit)
      |       if ~strcmp(fltLowerLimit_bkup,'0')
      |         set_param(gcb,'fltLowerLimit','0');
      |       end
      |     else
      |       tmps=num2str(fltLowerLimit);
      |       if ~strcmp(fltLowerLimit_bkup,tmps)
      |         set_param(gcb,'fltLowerLimit',tmps);
      |       end
      |     end
      |     if isnan(fltUpperLimit)
      |       if ~strcmp(fltUpperLimit_bkup,'0')
      |         set_param(gcb,'fltUpperLimit','0');
      |       end
      |     else
      |       tmps=num2str(fltUpperLimit);
      |       if ~strcmp(fltUpperLimit_bkup,tmps)
      |         set_param(gcb,'fltUpperLimit',tmps);
      |       end
      |     end
      |   end
      | end
      mask Callback wf0:
      | autoCalcEn=get_param(gcb,'autoCalcEn');
      | if strcmp(autoCalcEn,'on')
      |   SampleTime=Simulink.data.evalinGlobal(bdroot,get_param(gcb,'SampleTime'));
      |   if (SampleTime==-1)
      |     SampleTime=str2double(get_param(gcb,'SampleTime_1'));
      |   end
      |   fltUmaxDivImax_bkup=get_param(gcb,'fltUmaxDivImax');
      |   fltLambda_bkup=get_param(gcb,'fltLambda');
      |   fltPropGain_bkup=get_param(gcb,'fltPropGain');
      |   fltIntegGain_bkup=get_param(gcb,'fltIntegGain');
      |   fltLowerLimit_bkup=get_param(gcb,'fltLowerLimit');
      |   fltUpperLimit_bkup=get_param(gcb,'fltUpperLimit');
      |   wf0=Simulink.data.evalinGlobal(bdroot,get_param(gcb,'wf0'));
      |   wksi=Simulink.data.evalinGlobal(bdroot,get_param(gcb,'wksi'));
      |   J=Simulink.data.evalinGlobal(bdroot,get_param(gcb,'J'));
      |   Kt=Simulink.data.evalinGlobal(bdroot,get_param(gcb,'Kt'));
      |   lambdaFW=Simulink.data.evalinGlobal(bdroot,get_param(gcb,'lambdaFW'));
      |   Idmax=Simulink.data.evalinGlobal(bdroot,get_param(gcb,'Idmax'));
      |   imax=Simulink.data.evalinGlobal(bdroot,get_param(gcb,'imax'));
      |   udcbus=Simulink.data.evalinGlobal(bdroot,get_param(gcb,'udcbus'));
      |   if (wf0<=0)
      |     warning('Natural frequency f0 must be positive.');
      |   end
      |   if (wksi<=0)
      |     warning('Current loop attenuation must be positive.');
      |   end
      |   if (wksi>1)
      |     warning('Current loop attenuation must not exceed 1.');
      |   end
      |   if (J<=0)
      |     warning('Moment of inertia J must be positive.');
      |   end
      |   if (Kt<=0)
      |     warning('Torque constant Kt must be positive.');
      |   end
      |   if (lambdaFW<0)
      |     warning('MA filter smoothing factor must be in the range 0..1.');
      |   end
      |   if (lambdaFW>1)
      |     warning('MA filter smoothing factor must be in the range 0..1.');
      |   end
      |   if (udcbus<=0)
      |     warning('DC bus voltage must be positive.');
      |   end
      |   if (imax<=0)
      |     warning('Max. phase current must be positive.');
      |   end
      |   w0=6.283185307179586*wf0;
      |   pgain=2.0*wksi*w0*J/Kt;
      |   igain=w0*w0*J/Kt;
      |   fltPropGain=0.9*pgain;
      |   fltIntegGain=igain*SampleTime*0.5;
      |   if (Idmax<0)
      |     iratio=abs(Idmax)/imax;
      |     lowlim=acos(iratio)-1.570796326794897;
      |   else
      |     lowlim=0.0;
      |   end
      |   fltLowerLimit=lowlim;
      |   fltUpperLimit=0.0;
      |   fltLambda=lambdaFW;
      |   fltUmaxDivImax=0.5773502691896258*udcbus/imax;
      |   if isnan(fltUmaxDivImax)
      |     if ~strcmp(fltUmaxDivImax_bkup,'0')
      |       set_param(gcb,'fltUmaxDivImax','0');
      |     end
      |   else
      |     tmps=num2str(fltUmaxDivImax);
      |     if ~strcmp(fltUmaxDivImax_bkup,tmps)
      |       set_param(gcb,'fltUmaxDivImax',tmps);
      |     end
      |   end
      |   if isnan(fltLambda)
      |     if ~strcmp(fltLambda_bkup,'0')
      |       set_param(gcb,'fltLambda','0');
      |     end
      |   else
      |     tmps=num2str(fltLambda);
      |     if ~strcmp(fltLambda_bkup,tmps)
      |       set_param(gcb,'fltLambda',tmps);
      |     end
      |   end
      |   if isnan(fltPropGain)
      |     if ~strcmp(fltPropGain_bkup,'0')
      |       set_param(gcb,'fltPropGain','0');
      |     end
      |   else
      |     tmps=num2str(fltPropGain);
      |     if ~strcmp(fltPropGain_bkup,tmps)
      |       set_param(gcb,'fltPropGain',tmps);
      |     end
      |   end
      |   if isnan(fltIntegGain)
      |     if ~strcmp(fltIntegGain_bkup,'0')
      |       set_param(gcb,'fltIntegGain','0');
      |     end
      |   else
      |     tmps=num2str(fltIntegGain);
      |     if ~strcmp(fltIntegGain_bkup,tmps)
      |       set_param(gcb,'fltIntegGain',tmps);
      |     end
      |   end
      |   if isnan(fltLowerLimit)
      |     if ~strcmp(fltLowerLimit_bkup,'0')
      |       set_param(gcb,'fltLowerLimit','0');
      |     end
      |   else
      |     tmps=num2str(fltLowerLimit);
      |     if ~strcmp(fltLowerLimit_bkup,tmps)
      |       set_param(gcb,'fltLowerLimit',tmps);
      |     end
      |   end
      |   if isnan(fltUpperLimit)
      |     if ~strcmp(fltUpperLimit_bkup,'0')
      |       set_param(gcb,'fltUpperLimit','0');
      |     end
      |   else
      |     tmps=num2str(fltUpperLimit);
      |     if ~strcmp(fltUpperLimit_bkup,tmps)
      |       set_param(gcb,'fltUpperLimit',tmps);
      |     end
      |   end
      | end
      mask Callback wksi:
      | autoCalcEn=get_param(gcb,'autoCalcEn');
      | if strcmp(autoCalcEn,'on')
      |   SampleTime=Simulink.data.evalinGlobal(bdroot,get_param(gcb,'SampleTime'));
      |   if (SampleTime==-1)
      |     SampleTime=str2double(get_param(gcb,'SampleTime_1'));
      |   end
      |   fltUmaxDivImax_bkup=get_param(gcb,'fltUmaxDivImax');
      |   fltLambda_bkup=get_param(gcb,'fltLambda');
      |   fltPropGain_bkup=get_param(gcb,'fltPropGain');
      |   fltIntegGain_bkup=get_param(gcb,'fltIntegGain');
      |   fltLowerLimit_bkup=get_param(gcb,'fltLowerLimit');
      |   fltUpperLimit_bkup=get_param(gcb,'fltUpperLimit');
      |   wf0=Simulink.data.evalinGlobal(bdroot,get_param(gcb,'wf0'));
      |   wksi=Simulink.data.evalinGlobal(bdroot,get_param(gcb,'wksi'));
      |   J=Simulink.data.evalinGlobal(bdroot,get_param(gcb,'J'));
      |   Kt=Simulink.data.evalinGlobal(bdroot,get_param(gcb,'Kt'));
      |   lambdaFW=Simulink.data.evalinGlobal(bdroot,get_param(gcb,'lambdaFW'));
      |   Idmax=Simulink.data.evalinGlobal(bdroot,get_param(gcb,'Idmax'));
      |   imax=Simulink.data.evalinGlobal(bdroot,get_param(gcb,'imax'));
      |   udcbus=Simulink.data.evalinGlobal(bdroot,get_param(gcb,'udcbus'));
      |   if (wf0<=0)
      |     warning('Natural frequency f0 must be positive.');
      |   end
      |   if (wksi<=0)
      |     warning('Current loop attenuation must be positive.');
      |   end
      |   if (wksi>1)
      |     warning('Current loop attenuation must not exceed 1.');
      |   end
      |   if (J<=0)
      |     warning('Moment of inertia J must be positive.');
      |   end
      |   if (Kt<=0)
      |     warning('Torque constant Kt must be positive.');
      |   end
      |   if (lambdaFW<0)
      |     warning('MA filter smoothing factor must be in the range 0..1.');
      |   end
      |   if (lambdaFW>1)
      |     warning('MA filter smoothing factor must be in the range 0..1.');
      |   end
      |   if (udcbus<=0)
      |     warning('DC bus voltage must be positive.');
      |   end
      |   if (imax<=0)
      |     warning('Max. phase current must be positive.');
      |   end
      |   w0=6.283185307179586*wf0;
      |   pgain=2.0*wksi*w0*J/Kt;
      |   igain=w0*w0*J/Kt;
      |   fltPropGain=0.9*pgain;
      |   fltIntegGain=igain*SampleTime*0.5;
      |   if (Idmax<0)
      |     iratio=abs(Idmax)/imax;
      |     lowlim=acos(iratio)-1.570796326794897;
      |   else
      |     lowlim=0.0;
      |   end
      |   fltLowerLimit=lowlim;
      |   fltUpperLimit=0.0;
      |   fltLambda=lambdaFW;
      |   fltUmaxDivImax=0.5773502691896258*udcbus/imax;
      |   if isnan(fltUmaxDivImax)
      |     if ~strcmp(fltUmaxDivImax_bkup,'0')
      |       set_param(gcb,'fltUmaxDivImax','0');
      |     end
      |   else
      |     tmps=num2str(fltUmaxDivImax);
      |     if ~strcmp(fltUmaxDivImax_bkup,tmps)
      |       set_param(gcb,'fltUmaxDivImax',tmps);
      |     end
      |   end
      |   if isnan(fltLambda)
      |     if ~strcmp(fltLambda_bkup,'0')
      |       set_param(gcb,'fltLambda','0');
      |     end
      |   else
      |     tmps=num2str(fltLambda);
      |     if ~strcmp(fltLambda_bkup,tmps)
      |       set_param(gcb,'fltLambda',tmps);
      |     end
      |   end
      |   if isnan(fltPropGain)
      |     if ~strcmp(fltPropGain_bkup,'0')
      |       set_param(gcb,'fltPropGain','0');
      |     end
      |   else
      |     tmps=num2str(fltPropGain);
      |     if ~strcmp(fltPropGain_bkup,tmps)
      |       set_param(gcb,'fltPropGain',tmps);
      |     end
      |   end
      |   if isnan(fltIntegGain)
      |     if ~strcmp(fltIntegGain_bkup,'0')
      |       set_param(gcb,'fltIntegGain','0');
      |     end
      |   else
      |     tmps=num2str(fltIntegGain);
      |     if ~strcmp(fltIntegGain_bkup,tmps)
      |       set_param(gcb,'fltIntegGain',tmps);
      |     end
      |   end
      |   if isnan(fltLowerLimit)
      |     if ~strcmp(fltLowerLimit_bkup,'0')
      |       set_param(gcb,'fltLowerLimit','0');
      |     end
      |   else
      |     tmps=num2str(fltLowerLimit);
      |     if ~strcmp(fltLowerLimit_bkup,tmps)
      |       set_param(gcb,'fltLowerLimit',tmps);
      |     end
      |   end
      |   if isnan(fltUpperLimit)
      |     if ~strcmp(fltUpperLimit_bkup,'0')
      |       set_param(gcb,'fltUpperLimit','0');
      |     end
      |   else
      |     tmps=num2str(fltUpperLimit);
      |     if ~strcmp(fltUpperLimit_bkup,tmps)
      |       set_param(gcb,'fltUpperLimit',tmps);
      |     end
      |   end
      | end
      mask Callback J:
      | autoCalcEn=get_param(gcb,'autoCalcEn');
      | if strcmp(autoCalcEn,'on')
      |   SampleTime=Simulink.data.evalinGlobal(bdroot,get_param(gcb,'SampleTime'));
      |   if (SampleTime==-1)
      |     SampleTime=str2double(get_param(gcb,'SampleTime_1'));
      |   end
      |   fltUmaxDivImax_bkup=get_param(gcb,'fltUmaxDivImax');
      |   fltLambda_bkup=get_param(gcb,'fltLambda');
      |   fltPropGain_bkup=get_param(gcb,'fltPropGain');
      |   fltIntegGain_bkup=get_param(gcb,'fltIntegGain');
      |   fltLowerLimit_bkup=get_param(gcb,'fltLowerLimit');
      |   fltUpperLimit_bkup=get_param(gcb,'fltUpperLimit');
      |   wf0=Simulink.data.evalinGlobal(bdroot,get_param(gcb,'wf0'));
      |   wksi=Simulink.data.evalinGlobal(bdroot,get_param(gcb,'wksi'));
      |   J=Simulink.data.evalinGlobal(bdroot,get_param(gcb,'J'));
      |   Kt=Simulink.data.evalinGlobal(bdroot,get_param(gcb,'Kt'));
      |   lambdaFW=Simulink.data.evalinGlobal(bdroot,get_param(gcb,'lambdaFW'));
      |   Idmax=Simulink.data.evalinGlobal(bdroot,get_param(gcb,'Idmax'));
      |   imax=Simulink.data.evalinGlobal(bdroot,get_param(gcb,'imax'));
      |   udcbus=Simulink.data.evalinGlobal(bdroot,get_param(gcb,'udcbus'));
      |   if (wf0<=0)
      |     warning('Natural frequency f0 must be positive.');
      |   end
      |   if (wksi<=0)
      |     warning('Current loop attenuation must be positive.');
      |   end
      |   if (wksi>1)
      |     warning('Current loop attenuation must not exceed 1.');
      |   end
      |   if (J<=0)
      |     warning('Moment of inertia J must be positive.');
      |   end
      |   if (Kt<=0)
      |     warning('Torque constant Kt must be positive.');
      |   end
      |   if (lambdaFW<0)
      |     warning('MA filter smoothing factor must be in the range 0..1.');
      |   end
      |   if (lambdaFW>1)
      |     warning('MA filter smoothing factor must be in the range 0..1.');
      |   end
      |   if (udcbus<=0)
      |     warning('DC bus voltage must be positive.');
      |   end
      |   if (imax<=0)
      |     warning('Max. phase current must be positive.');
      |   end
      |   w0=6.283185307179586*wf0;
      |   pgain=2.0*wksi*w0*J/Kt;
      |   igain=w0*w0*J/Kt;
      |   fltPropGain=0.9*pgain;
      |   fltIntegGain=igain*SampleTime*0.5;
      |   if (Idmax<0)
      |     iratio=abs(Idmax)/imax;
      |     lowlim=acos(iratio)-1.570796326794897;
      |   else
      |     lowlim=0.0;
      |   end
      |   fltLowerLimit=lowlim;
      |   fltUpperLimit=0.0;
      |   fltLambda=lambdaFW;
      |   fltUmaxDivImax=0.5773502691896258*udcbus/imax;
      |   if isnan(fltUmaxDivImax)
      |     if ~strcmp(fltUmaxDivImax_bkup,'0')
      |       set_param(gcb,'fltUmaxDivImax','0');
      |     end
      |   else
      |     tmps=num2str(fltUmaxDivImax);
      |     if ~strcmp(fltUmaxDivImax_bkup,tmps)
      |       set_param(gcb,'fltUmaxDivImax',tmps);
      |     end
      |   end
      |   if isnan(fltLambda)
      |     if ~strcmp(fltLambda_bkup,'0')
      |       set_param(gcb,'fltLambda','0');
      |     end
      |   else
      |     tmps=num2str(fltLambda);
      |     if ~strcmp(fltLambda_bkup,tmps)
      |       set_param(gcb,'fltLambda',tmps);
      |     end
      |   end
      |   if isnan(fltPropGain)
      |     if ~strcmp(fltPropGain_bkup,'0')
      |       set_param(gcb,'fltPropGain','0');
      |     end
      |   else
      |     tmps=num2str(fltPropGain);
      |     if ~strcmp(fltPropGain_bkup,tmps)
      |       set_param(gcb,'fltPropGain',tmps);
      |     end
      |   end
      |   if isnan(fltIntegGain)
      |     if ~strcmp(fltIntegGain_bkup,'0')
      |       set_param(gcb,'fltIntegGain','0');
      |     end
      |   else
      |     tmps=num2str(fltIntegGain);
      |     if ~strcmp(fltIntegGain_bkup,tmps)
      |       set_param(gcb,'fltIntegGain',tmps);
      |     end
      |   end
      |   if isnan(fltLowerLimit)
      |     if ~strcmp(fltLowerLimit_bkup,'0')
      |       set_param(gcb,'fltLowerLimit','0');
      |     end
      |   else
      |     tmps=num2str(fltLowerLimit);
      |     if ~strcmp(fltLowerLimit_bkup,tmps)
      |       set_param(gcb,'fltLowerLimit',tmps);
      |     end
      |   end
      |   if isnan(fltUpperLimit)
      |     if ~strcmp(fltUpperLimit_bkup,'0')
      |       set_param(gcb,'fltUpperLimit','0');
      |     end
      |   else
      |     tmps=num2str(fltUpperLimit);
      |     if ~strcmp(fltUpperLimit_bkup,tmps)
      |       set_param(gcb,'fltUpperLimit',tmps);
      |     end
      |   end
      | end
      mask Callback Kt:
      | autoCalcEn=get_param(gcb,'autoCalcEn');
      | if strcmp(autoCalcEn,'on')
      |   SampleTime=Simulink.data.evalinGlobal(bdroot,get_param(gcb,'SampleTime'));
      |   if (SampleTime==-1)
      |     SampleTime=str2double(get_param(gcb,'SampleTime_1'));
      |   end
      |   fltUmaxDivImax_bkup=get_param(gcb,'fltUmaxDivImax');
      |   fltLambda_bkup=get_param(gcb,'fltLambda');
      |   fltPropGain_bkup=get_param(gcb,'fltPropGain');
      |   fltIntegGain_bkup=get_param(gcb,'fltIntegGain');
      |   fltLowerLimit_bkup=get_param(gcb,'fltLowerLimit');
      |   fltUpperLimit_bkup=get_param(gcb,'fltUpperLimit');
      |   wf0=Simulink.data.evalinGlobal(bdroot,get_param(gcb,'wf0'));
      |   wksi=Simulink.data.evalinGlobal(bdroot,get_param(gcb,'wksi'));
      |   J=Simulink.data.evalinGlobal(bdroot,get_param(gcb,'J'));
      |   Kt=Simulink.data.evalinGlobal(bdroot,get_param(gcb,'Kt'));
      |   lambdaFW=Simulink.data.evalinGlobal(bdroot,get_param(gcb,'lambdaFW'));
      |   Idmax=Simulink.data.evalinGlobal(bdroot,get_param(gcb,'Idmax'));
      |   imax=Simulink.data.evalinGlobal(bdroot,get_param(gcb,'imax'));
      |   udcbus=Simulink.data.evalinGlobal(bdroot,get_param(gcb,'udcbus'));
      |   if (wf0<=0)
      |     warning('Natural frequency f0 must be positive.');
      |   end
      |   if (wksi<=0)
      |     warning('Current loop attenuation must be positive.');
      |   end
      |   if (wksi>1)
      |     warning('Current loop attenuation must not exceed 1.');
      |   end
      |   if (J<=0)
      |     warning('Moment of inertia J must be positive.');
      |   end
      |   if (Kt<=0)
      |     warning('Torque constant Kt must be positive.');
      |   end
      |   if (lambdaFW<0)
      |     warning('MA filter smoothing factor must be in the range 0..1.');
      |   end
      |   if (lambdaFW>1)
      |     warning('MA filter smoothing factor must be in the range 0..1.');
      |   end
      |   if (udcbus<=0)
      |     warning('DC bus voltage must be positive.');
      |   end
      |   if (imax<=0)
      |     warning('Max. phase current must be positive.');
      |   end
      |   w0=6.283185307179586*wf0;
      |   pgain=2.0*wksi*w0*J/Kt;
      |   igain=w0*w0*J/Kt;
      |   fltPropGain=0.9*pgain;
      |   fltIntegGain=igain*SampleTime*0.5;
      |   if (Idmax<0)
      |     iratio=abs(Idmax)/imax;
      |     lowlim=acos(iratio)-1.570796326794897;
      |   else
      |     lowlim=0.0;
      |   end
      |   fltLowerLimit=lowlim;
      |   fltUpperLimit=0.0;
      |   fltLambda=lambdaFW;
      |   fltUmaxDivImax=0.5773502691896258*udcbus/imax;
      |   if isnan(fltUmaxDivImax)
      |     if ~strcmp(fltUmaxDivImax_bkup,'0')
      |       set_param(gcb,'fltUmaxDivImax','0');
      |     end
      |   else
      |     tmps=num2str(fltUmaxDivImax);
      |     if ~strcmp(fltUmaxDivImax_bkup,tmps)
      |       set_param(gcb,'fltUmaxDivImax',tmps);
      |     end
      |   end
      |   if isnan(fltLambda)
      |     if ~strcmp(fltLambda_bkup,'0')
      |       set_param(gcb,'fltLambda','0');
      |     end
      |   else
      |     tmps=num2str(fltLambda);
      |     if ~strcmp(fltLambda_bkup,tmps)
      |       set_param(gcb,'fltLambda',tmps);
      |     end
      |   end
      |   if isnan(fltPropGain)
      |     if ~strcmp(fltPropGain_bkup,'0')
      |       set_param(gcb,'fltPropGain','0');
      |     end
      |   else
      |     tmps=num2str(fltPropGain);
      |     if ~strcmp(fltPropGain_bkup,tmps)
      |       set_param(gcb,'fltPropGain',tmps);
      |     end
      |   end
      |   if isnan(fltIntegGain)
      |     if ~strcmp(fltIntegGain_bkup,'0')
      |       set_param(gcb,'fltIntegGain','0');
      |     end
      |   else
      |     tmps=num2str(fltIntegGain);
      |     if ~strcmp(fltIntegGain_bkup,tmps)
      |       set_param(gcb,'fltIntegGain',tmps);
      |     end
      |   end
      |   if isnan(fltLowerLimit)
      |     if ~strcmp(fltLowerLimit_bkup,'0')
      |       set_param(gcb,'fltLowerLimit','0');
      |     end
      |   else
      |     tmps=num2str(fltLowerLimit);
      |     if ~strcmp(fltLowerLimit_bkup,tmps)
      |       set_param(gcb,'fltLowerLimit',tmps);
      |     end
      |   end
      |   if isnan(fltUpperLimit)
      |     if ~strcmp(fltUpperLimit_bkup,'0')
      |       set_param(gcb,'fltUpperLimit','0');
      |     end
      |   else
      |     tmps=num2str(fltUpperLimit);
      |     if ~strcmp(fltUpperLimit_bkup,tmps)
      |       set_param(gcb,'fltUpperLimit',tmps);
      |     end
      |   end
      | end
      mask Callback lambdaFW:
      | autoCalcEn=get_param(gcb,'autoCalcEn');
      | if strcmp(autoCalcEn,'on')
      |   SampleTime=Simulink.data.evalinGlobal(bdroot,get_param(gcb,'SampleTime'));
      |   if (SampleTime==-1)
      |     SampleTime=str2double(get_param(gcb,'SampleTime_1'));
      |   end
      |   fltUmaxDivImax_bkup=get_param(gcb,'fltUmaxDivImax');
      |   fltLambda_bkup=get_param(gcb,'fltLambda');
      |   fltPropGain_bkup=get_param(gcb,'fltPropGain');
      |   fltIntegGain_bkup=get_param(gcb,'fltIntegGain');
      |   fltLowerLimit_bkup=get_param(gcb,'fltLowerLimit');
      |   fltUpperLimit_bkup=get_param(gcb,'fltUpperLimit');
      |   wf0=Simulink.data.evalinGlobal(bdroot,get_param(gcb,'wf0'));
      |   wksi=Simulink.data.evalinGlobal(bdroot,get_param(gcb,'wksi'));
      |   J=Simulink.data.evalinGlobal(bdroot,get_param(gcb,'J'));
      |   Kt=Simulink.data.evalinGlobal(bdroot,get_param(gcb,'Kt'));
      |   lambdaFW=Simulink.data.evalinGlobal(bdroot,get_param(gcb,'lambdaFW'));
      |   Idmax=Simulink.data.evalinGlobal(bdroot,get_param(gcb,'Idmax'));
      |   imax=Simulink.data.evalinGlobal(bdroot,get_param(gcb,'imax'));
      |   udcbus=Simulink.data.evalinGlobal(bdroot,get_param(gcb,'udcbus'));
      |   if (wf0<=0)
      |     warning('Natural frequency f0 must be positive.');
      |   end
      |   if (wksi<=0)
      |     warning('Current loop attenuation must be positive.');
      |   end
      |   if (wksi>1)
      |     warning('Current loop attenuation must not exceed 1.');
      |   end
      |   if (J<=0)
      |     warning('Moment of inertia J must be positive.');
      |   end
      |   if (Kt<=0)
      |     warning('Torque constant Kt must be positive.');
      |   end
      |   if (lambdaFW<0)
      |     warning('MA filter smoothing factor must be in the range 0..1.');
      |   end
      |   if (lambdaFW>1)
      |     warning('MA filter smoothing factor must be in the range 0..1.');
      |   end
      |   if (udcbus<=0)
      |     warning('DC bus voltage must be positive.');
      |   end
      |   if (imax<=0)
      |     warning('Max. phase current must be positive.');
      |   end
      |   w0=6.283185307179586*wf0;
      |   pgain=2.0*wksi*w0*J/Kt;
      |   igain=w0*w0*J/Kt;
      |   fltPropGain=0.9*pgain;
      |   fltIntegGain=igain*SampleTime*0.5;
      |   if (Idmax<0)
      |     iratio=abs(Idmax)/imax;
      |     lowlim=acos(iratio)-1.570796326794897;
      |   else
      |     lowlim=0.0;
      |   end
      |   fltLowerLimit=lowlim;
      |   fltUpperLimit=0.0;
      |   fltLambda=lambdaFW;
      |   fltUmaxDivImax=0.5773502691896258*udcbus/imax;
      |   if isnan(fltUmaxDivImax)
      |     if ~strcmp(fltUmaxDivImax_bkup,'0')
      |       set_param(gcb,'fltUmaxDivImax','0');
      |     end
      |   else
      |     tmps=num2str(fltUmaxDivImax);
      |     if ~strcmp(fltUmaxDivImax_bkup,tmps)
      |       set_param(gcb,'fltUmaxDivImax',tmps);
      |     end
      |   end
      |   if isnan(fltLambda)
      |     if ~strcmp(fltLambda_bkup,'0')
      |       set_param(gcb,'fltLambda','0');
      |     end
      |   else
      |     tmps=num2str(fltLambda);
      |     if ~strcmp(fltLambda_bkup,tmps)
      |       set_param(gcb,'fltLambda',tmps);
      |     end
      |   end
      |   if isnan(fltPropGain)
      |     if ~strcmp(fltPropGain_bkup,'0')
      |       set_param(gcb,'fltPropGain','0');
      |     end
      |   else
      |     tmps=num2str(fltPropGain);
      |     if ~strcmp(fltPropGain_bkup,tmps)
      |       set_param(gcb,'fltPropGain',tmps);
      |     end
      |   end
      |   if isnan(fltIntegGain)
      |     if ~strcmp(fltIntegGain_bkup,'0')
      |       set_param(gcb,'fltIntegGain','0');
      |     end
      |   else
      |     tmps=num2str(fltIntegGain);
      |     if ~strcmp(fltIntegGain_bkup,tmps)
      |       set_param(gcb,'fltIntegGain',tmps);
      |     end
      |   end
      |   if isnan(fltLowerLimit)
      |     if ~strcmp(fltLowerLimit_bkup,'0')
      |       set_param(gcb,'fltLowerLimit','0');
      |     end
      |   else
      |     tmps=num2str(fltLowerLimit);
      |     if ~strcmp(fltLowerLimit_bkup,tmps)
      |       set_param(gcb,'fltLowerLimit',tmps);
      |     end
      |   end
      |   if isnan(fltUpperLimit)
      |     if ~strcmp(fltUpperLimit_bkup,'0')
      |       set_param(gcb,'fltUpperLimit','0');
      |     end
      |   else
      |     tmps=num2str(fltUpperLimit);
      |     if ~strcmp(fltUpperLimit_bkup,tmps)
      |       set_param(gcb,'fltUpperLimit',tmps);
      |     end
      |   end
      | end
      mask Callback Idmax:
      | autoCalcEn=get_param(gcb,'autoCalcEn');
      | if strcmp(autoCalcEn,'on')
      |   SampleTime=Simulink.data.evalinGlobal(bdroot,get_param(gcb,'SampleTime'));
      |   if (SampleTime==-1)
      |     SampleTime=str2double(get_param(gcb,'SampleTime_1'));
      |   end
      |   fltUmaxDivImax_bkup=get_param(gcb,'fltUmaxDivImax');
      |   fltLambda_bkup=get_param(gcb,'fltLambda');
      |   fltPropGain_bkup=get_param(gcb,'fltPropGain');
      |   fltIntegGain_bkup=get_param(gcb,'fltIntegGain');
      |   fltLowerLimit_bkup=get_param(gcb,'fltLowerLimit');
      |   fltUpperLimit_bkup=get_param(gcb,'fltUpperLimit');
      |   wf0=Simulink.data.evalinGlobal(bdroot,get_param(gcb,'wf0'));
      |   wksi=Simulink.data.evalinGlobal(bdroot,get_param(gcb,'wksi'));
      |   J=Simulink.data.evalinGlobal(bdroot,get_param(gcb,'J'));
      |   Kt=Simulink.data.evalinGlobal(bdroot,get_param(gcb,'Kt'));
      |   lambdaFW=Simulink.data.evalinGlobal(bdroot,get_param(gcb,'lambdaFW'));
      |   Idmax=Simulink.data.evalinGlobal(bdroot,get_param(gcb,'Idmax'));
      |   imax=Simulink.data.evalinGlobal(bdroot,get_param(gcb,'imax'));
      |   udcbus=Simulink.data.evalinGlobal(bdroot,get_param(gcb,'udcbus'));
      |   if (wf0<=0)
      |     warning('Natural frequency f0 must be positive.');
      |   end
      |   if (wksi<=0)
      |     warning('Current loop attenuation must be positive.');
      |   end
      |   if (wksi>1)
      |     warning('Current loop attenuation must not exceed 1.');
      |   end
      |   if (J<=0)
      |     warning('Moment of inertia J must be positive.');
      |   end
      |   if (Kt<=0)
      |     warning('Torque constant Kt must be positive.');
      |   end
      |   if (lambdaFW<0)
      |     warning('MA filter smoothing factor must be in the range 0..1.');
      |   end
      |   if (lambdaFW>1)
      |     warning('MA filter smoothing factor must be in the range 0..1.');
      |   end
      |   if (udcbus<=0)
      |     warning('DC bus voltage must be positive.');
      |   end
      |   if (imax<=0)
      |     warning('Max. phase current must be positive.');
      |   end
      |   w0=6.283185307179586*wf0;
      |   pgain=2.0*wksi*w0*J/Kt;
      |   igain=w0*w0*J/Kt;
      |   fltPropGain=0.9*pgain;
      |   fltIntegGain=igain*SampleTime*0.5;
      |   if (Idmax<0)
      |     iratio=abs(Idmax)/imax;
      |     lowlim=acos(iratio)-1.570796326794897;
      |   else
      |     lowlim=0.0;
      |   end
      |   fltLowerLimit=lowlim;
      |   fltUpperLimit=0.0;
      |   fltLambda=lambdaFW;
      |   fltUmaxDivImax=0.5773502691896258*udcbus/imax;
      |   if isnan(fltUmaxDivImax)
      |     if ~strcmp(fltUmaxDivImax_bkup,'0')
      |       set_param(gcb,'fltUmaxDivImax','0');
      |     end
      |   else
      |     tmps=num2str(fltUmaxDivImax);
      |     if ~strcmp(fltUmaxDivImax_bkup,tmps)
      |       set_param(gcb,'fltUmaxDivImax',tmps);
      |     end
      |   end
      |   if isnan(fltLambda)
      |     if ~strcmp(fltLambda_bkup,'0')
      |       set_param(gcb,'fltLambda','0');
      |     end
      |   else
      |     tmps=num2str(fltLambda);
      |     if ~strcmp(fltLambda_bkup,tmps)
      |       set_param(gcb,'fltLambda',tmps);
      |     end
      |   end
      |   if isnan(fltPropGain)
      |     if ~strcmp(fltPropGain_bkup,'0')
      |       set_param(gcb,'fltPropGain','0');
      |     end
      |   else
      |     tmps=num2str(fltPropGain);
      |     if ~strcmp(fltPropGain_bkup,tmps)
      |       set_param(gcb,'fltPropGain',tmps);
      |     end
      |   end
      |   if isnan(fltIntegGain)
      |     if ~strcmp(fltIntegGain_bkup,'0')
      |       set_param(gcb,'fltIntegGain','0');
      |     end
      |   else
      |     tmps=num2str(fltIntegGain);
      |     if ~strcmp(fltIntegGain_bkup,tmps)
      |       set_param(gcb,'fltIntegGain',tmps);
      |     end
      |   end
      |   if isnan(fltLowerLimit)
      |     if ~strcmp(fltLowerLimit_bkup,'0')
      |       set_param(gcb,'fltLowerLimit','0');
      |     end
      |   else
      |     tmps=num2str(fltLowerLimit);
      |     if ~strcmp(fltLowerLimit_bkup,tmps)
      |       set_param(gcb,'fltLowerLimit',tmps);
      |     end
      |   end
      |   if isnan(fltUpperLimit)
      |     if ~strcmp(fltUpperLimit_bkup,'0')
      |       set_param(gcb,'fltUpperLimit','0');
      |     end
      |   else
      |     tmps=num2str(fltUpperLimit);
      |     if ~strcmp(fltUpperLimit_bkup,tmps)
      |       set_param(gcb,'fltUpperLimit',tmps);
      |     end
      |   end
      | end
      mask Callback imax:
      | autoCalcEn=get_param(gcb,'autoCalcEn');
      | if strcmp(autoCalcEn,'on')
      |   SampleTime=Simulink.data.evalinGlobal(bdroot,get_param(gcb,'SampleTime'));
      |   if (SampleTime==-1)
      |     SampleTime=str2double(get_param(gcb,'SampleTime_1'));
      |   end
      |   fltUmaxDivImax_bkup=get_param(gcb,'fltUmaxDivImax');
      |   fltLambda_bkup=get_param(gcb,'fltLambda');
      |   fltPropGain_bkup=get_param(gcb,'fltPropGain');
      |   fltIntegGain_bkup=get_param(gcb,'fltIntegGain');
      |   fltLowerLimit_bkup=get_param(gcb,'fltLowerLimit');
      |   fltUpperLimit_bkup=get_param(gcb,'fltUpperLimit');
      |   wf0=Simulink.data.evalinGlobal(bdroot,get_param(gcb,'wf0'));
      |   wksi=Simulink.data.evalinGlobal(bdroot,get_param(gcb,'wksi'));
      |   J=Simulink.data.evalinGlobal(bdroot,get_param(gcb,'J'));
      |   Kt=Simulink.data.evalinGlobal(bdroot,get_param(gcb,'Kt'));
      |   lambdaFW=Simulink.data.evalinGlobal(bdroot,get_param(gcb,'lambdaFW'));
      |   Idmax=Simulink.data.evalinGlobal(bdroot,get_param(gcb,'Idmax'));
      |   imax=Simulink.data.evalinGlobal(bdroot,get_param(gcb,'imax'));
      |   udcbus=Simulink.data.evalinGlobal(bdroot,get_param(gcb,'udcbus'));
      |   if (wf0<=0)
      |     warning('Natural frequency f0 must be positive.');
      |   end
      |   if (wksi<=0)
      |     warning('Current loop attenuation must be positive.');
      |   end
      |   if (wksi>1)
      |     warning('Current loop attenuation must not exceed 1.');
      |   end
      |   if (J<=0)
      |     warning('Moment of inertia J must be positive.');
      |   end
      |   if (Kt<=0)
      |     warning('Torque constant Kt must be positive.');
      |   end
      |   if (lambdaFW<0)
      |     warning('MA filter smoothing factor must be in the range 0..1.');
      |   end
      |   if (lambdaFW>1)
      |     warning('MA filter smoothing factor must be in the range 0..1.');
      |   end
      |   if (udcbus<=0)
      |     warning('DC bus voltage must be positive.');
      |   end
      |   if (imax<=0)
      |     warning('Max. phase current must be positive.');
      |   end
      |   w0=6.283185307179586*wf0;
      |   pgain=2.0*wksi*w0*J/Kt;
      |   igain=w0*w0*J/Kt;
      |   fltPropGain=0.9*pgain;
      |   fltIntegGain=igain*SampleTime*0.5;
      |   if (Idmax<0)
      |     iratio=abs(Idmax)/imax;
      |     lowlim=acos(iratio)-1.570796326794897;
      |   else
      |     lowlim=0.0;
      |   end
      |   fltLowerLimit=lowlim;
      |   fltUpperLimit=0.0;
      |   fltLambda=lambdaFW;
      |   fltUmaxDivImax=0.5773502691896258*udcbus/imax;
      |   if isnan(fltUmaxDivImax)
      |     if ~strcmp(fltUmaxDivImax_bkup,'0')
      |       set_param(gcb,'fltUmaxDivImax','0');
      |     end
      |   else
      |     tmps=num2str(fltUmaxDivImax);
      |     if ~strcmp(fltUmaxDivImax_bkup,tmps)
      |       set_param(gcb,'fltUmaxDivImax',tmps);
      |     end
      |   end
      |   if isnan(fltLambda)
      |     if ~strcmp(fltLambda_bkup,'0')
      |       set_param(gcb,'fltLambda','0');
      |     end
      |   else
      |     tmps=num2str(fltLambda);
      |     if ~strcmp(fltLambda_bkup,tmps)
      |       set_param(gcb,'fltLambda',tmps);
      |     end
      |   end
      |   if isnan(fltPropGain)
      |     if ~strcmp(fltPropGain_bkup,'0')
      |       set_param(gcb,'fltPropGain','0');
      |     end
      |   else
      |     tmps=num2str(fltPropGain);
      |     if ~strcmp(fltPropGain_bkup,tmps)
      |       set_param(gcb,'fltPropGain',tmps);
      |     end
      |   end
      |   if isnan(fltIntegGain)
      |     if ~strcmp(fltIntegGain_bkup,'0')
      |       set_param(gcb,'fltIntegGain','0');
      |     end
      |   else
      |     tmps=num2str(fltIntegGain);
      |     if ~strcmp(fltIntegGain_bkup,tmps)
      |       set_param(gcb,'fltIntegGain',tmps);
      |     end
      |   end
      |   if isnan(fltLowerLimit)
      |     if ~strcmp(fltLowerLimit_bkup,'0')
      |       set_param(gcb,'fltLowerLimit','0');
      |     end
      |   else
      |     tmps=num2str(fltLowerLimit);
      |     if ~strcmp(fltLowerLimit_bkup,tmps)
      |       set_param(gcb,'fltLowerLimit',tmps);
      |     end
      |   end
      |   if isnan(fltUpperLimit)
      |     if ~strcmp(fltUpperLimit_bkup,'0')
      |       set_param(gcb,'fltUpperLimit','0');
      |     end
      |   else
      |     tmps=num2str(fltUpperLimit);
      |     if ~strcmp(fltUpperLimit_bkup,tmps)
      |       set_param(gcb,'fltUpperLimit',tmps);
      |     end
      |   end
      | end
      mask Callback udcbus:
      | autoCalcEn=get_param(gcb,'autoCalcEn');
      | if strcmp(autoCalcEn,'on')
      |   SampleTime=Simulink.data.evalinGlobal(bdroot,get_param(gcb,'SampleTime'));
      |   if (SampleTime==-1)
      |     SampleTime=str2double(get_param(gcb,'SampleTime_1'));
      |   end
      |   fltUmaxDivImax_bkup=get_param(gcb,'fltUmaxDivImax');
      |   fltLambda_bkup=get_param(gcb,'fltLambda');
      |   fltPropGain_bkup=get_param(gcb,'fltPropGain');
      |   fltIntegGain_bkup=get_param(gcb,'fltIntegGain');
      |   fltLowerLimit_bkup=get_param(gcb,'fltLowerLimit');
      |   fltUpperLimit_bkup=get_param(gcb,'fltUpperLimit');
      |   wf0=Simulink.data.evalinGlobal(bdroot,get_param(gcb,'wf0'));
      |   wksi=Simulink.data.evalinGlobal(bdroot,get_param(gcb,'wksi'));
      |   J=Simulink.data.evalinGlobal(bdroot,get_param(gcb,'J'));
      |   Kt=Simulink.data.evalinGlobal(bdroot,get_param(gcb,'Kt'));
      |   lambdaFW=Simulink.data.evalinGlobal(bdroot,get_param(gcb,'lambdaFW'));
      |   Idmax=Simulink.data.evalinGlobal(bdroot,get_param(gcb,'Idmax'));
      |   imax=Simulink.data.evalinGlobal(bdroot,get_param(gcb,'imax'));
      |   udcbus=Simulink.data.evalinGlobal(bdroot,get_param(gcb,'udcbus'));
      |   if (wf0<=0)
      |     warning('Natural frequency f0 must be positive.');
      |   end
      |   if (wksi<=0)
      |     warning('Current loop attenuation must be positive.');
      |   end
      |   if (wksi>1)
      |     warning('Current loop attenuation must not exceed 1.');
      |   end
      |   if (J<=0)
      |     warning('Moment of inertia J must be positive.');
      |   end
      |   if (Kt<=0)
      |     warning('Torque constant Kt must be positive.');
      |   end
      |   if (lambdaFW<0)
      |     warning('MA filter smoothing factor must be in the range 0..1.');
      |   end
      |   if (lambdaFW>1)
      |     warning('MA filter smoothing factor must be in the range 0..1.');
      |   end
      |   if (udcbus<=0)
      |     warning('DC bus voltage must be positive.');
      |   end
      |   if (imax<=0)
      |     warning('Max. phase current must be positive.');
      |   end
      |   w0=6.283185307179586*wf0;
      |   pgain=2.0*wksi*w0*J/Kt;
      |   igain=w0*w0*J/Kt;
      |   fltPropGain=0.9*pgain;
      |   fltIntegGain=igain*SampleTime*0.5;
      |   if (Idmax<0)
      |     iratio=abs(Idmax)/imax;
      |     lowlim=acos(iratio)-1.570796326794897;
      |   else
      |     lowlim=0.0;
      |   end
      |   fltLowerLimit=lowlim;
      |   fltUpperLimit=0.0;
      |   fltLambda=lambdaFW;
      |   fltUmaxDivImax=0.5773502691896258*udcbus/imax;
      |   if isnan(fltUmaxDivImax)
      |     if ~strcmp(fltUmaxDivImax_bkup,'0')
      |       set_param(gcb,'fltUmaxDivImax','0');
      |     end
      |   else
      |     tmps=num2str(fltUmaxDivImax);
      |     if ~strcmp(fltUmaxDivImax_bkup,tmps)
      |       set_param(gcb,'fltUmaxDivImax',tmps);
      |     end
      |   end
      |   if isnan(fltLambda)
      |     if ~strcmp(fltLambda_bkup,'0')
      |       set_param(gcb,'fltLambda','0');
      |     end
      |   else
      |     tmps=num2str(fltLambda);
      |     if ~strcmp(fltLambda_bkup,tmps)
      |       set_param(gcb,'fltLambda',tmps);
      |     end
      |   end
      |   if isnan(fltPropGain)
      |     if ~strcmp(fltPropGain_bkup,'0')
      |       set_param(gcb,'fltPropGain','0');
      |     end
      |   else
      |     tmps=num2str(fltPropGain);
      |     if ~strcmp(fltPropGain_bkup,tmps)
      |       set_param(gcb,'fltPropGain',tmps);
      |     end
      |   end
      |   if isnan(fltIntegGain)
      |     if ~strcmp(fltIntegGain_bkup,'0')
      |       set_param(gcb,'fltIntegGain','0');
      |     end
      |   else
      |     tmps=num2str(fltIntegGain);
      |     if ~strcmp(fltIntegGain_bkup,tmps)
      |       set_param(gcb,'fltIntegGain',tmps);
      |     end
      |   end
      |   if isnan(fltLowerLimit)
      |     if ~strcmp(fltLowerLimit_bkup,'0')
      |       set_param(gcb,'fltLowerLimit','0');
      |     end
      |   else
      |     tmps=num2str(fltLowerLimit);
      |     if ~strcmp(fltLowerLimit_bkup,tmps)
      |       set_param(gcb,'fltLowerLimit',tmps);
      |     end
      |   end
      |   if isnan(fltUpperLimit)
      |     if ~strcmp(fltUpperLimit_bkup,'0')
      |       set_param(gcb,'fltUpperLimit','0');
      |     end
      |   else
      |     tmps=num2str(fltUpperLimit);
      |     if ~strcmp(fltUpperLimit_bkup,tmps)
      |       set_param(gcb,'fltUpperLimit',tmps);
      |     end
      |   end
      | end
      mask Callback autoCalcEn:
      | maskStr=get_param(gcb,'showStates');
      | if strcmp(maskStr,'Hide (faster execution)')
      |   p=Simulink.Mask.get(gcb);
      |   autoCalcEn=get_param(gcb,'autoCalcEn');
      |   hintText=p.getDialogControl('timeHint');
      |   if strcmp(autoCalcEn,'on')
      |     param=p.getParameter('udcbus');
      |     if strcmp(param.Enabled,'off')
      |       SampleTime=Simulink.data.evalinGlobal(bdroot,get_param(gcb,'SampleTime'));
      |       if SampleTime==-1
      |         SampleTime=str2double(get_param(gcb,'SampleTime_1'));
      |         if isnan(SampleTime)
      |           hintText.Prompt=['Note: Implementation parameters cannot be calculated yet because the block''s inherited sample time is unknown. Simulink will update the sample time when you run the simulation.'];
      |         else
      |           hintText.Prompt=['Caution: Implementation parameters depend on inherited sample time. Make sure that the sample time of the block''s inputs corresponds to the sampling period in the target application.'];
      |         end
      |       else
      |         hintText.Prompt='Caution: Implementation parameters depend on the sample time. Make sure that the simulation time step corresponds to the sampling period in the target application.';
      |       end
      |       p=Simulink.Mask.get(gcb);
      |       param=p.getParameter('wf0');
      |       param.set('Enabled','on');
      |       param=p.getParameter('wksi');
      |       param.set('Enabled','on');
      |       param=p.getParameter('J');
      |       param.set('Enabled','on');
      |       param=p.getParameter('Kt');
      |       param.set('Enabled','on');
      |       param=p.getParameter('lambdaFW');
      |       param.set('Enabled','on');
      |       param=p.getParameter('Idmax');
      |       param.set('Enabled','on');
      |       param=p.getParameter('imax');
      |       param.set('Enabled','on');
      |       param=p.getParameter('udcbus');
      |       param.set('Enabled','on');
      |     else
      |       SampleTime=Simulink.data.evalinGlobal(bdroot,get_param(gcb,'SampleTime'));
      |       if SampleTime==-1
      |         SampleTime=str2double(get_param(gcb,'SampleTime_1'));
      |       end
      |     end
      |     fltUmaxDivImax_bkup=get_param(gcb,'fltUmaxDivImax');
      |     fltLambda_bkup=get_param(gcb,'fltLambda');
      |     fltPropGain_bkup=get_param(gcb,'fltPropGain');
      |     fltIntegGain_bkup=get_param(gcb,'fltIntegGain');
      |     fltLowerLimit_bkup=get_param(gcb,'fltLowerLimit');
      |     fltUpperLimit_bkup=get_param(gcb,'fltUpperLimit');
      |     wf0=Simulink.data.evalinGlobal(bdroot,get_param(gcb,'wf0'));
      |     wksi=Simulink.data.evalinGlobal(bdroot,get_param(gcb,'wksi'));
      |     J=Simulink.data.evalinGlobal(bdroot,get_param(gcb,'J'));
      |     Kt=Simulink.data.evalinGlobal(bdroot,get_param(gcb,'Kt'));
      |     lambdaFW=Simulink.data.evalinGlobal(bdroot,get_param(gcb,'lambdaFW'));
      |     Idmax=Simulink.data.evalinGlobal(bdroot,get_param(gcb,'Idmax'));
      |     imax=Simulink.data.evalinGlobal(bdroot,get_param(gcb,'imax'));
      |     udcbus=Simulink.data.evalinGlobal(bdroot,get_param(gcb,'udcbus'));
      |     if (wf0<=0)
      |       warning('Natural frequency f0 must be positive.');
      |     end
      |     if (wksi<=0)
      |       warning('Current loop attenuation must be positive.');
      |     end
      |     if (wksi>1)
      |       warning('Current loop attenuation must not exceed 1.');
      |     end
      |     if (J<=0)
      |       warning('Moment of inertia J must be positive.');
      |     end
      |     if (Kt<=0)
      |       warning('Torque constant Kt must be positive.');
      |     end
      |     if (lambdaFW<0)
      |       warning('MA filter smoothing factor must be in the range 0..1.');
      |     end
      |     if (lambdaFW>1)
      |       warning('MA filter smoothing factor must be in the range 0..1.');
      |     end
      |     if (udcbus<=0)
      |       warning('DC bus voltage must be positive.');
      |     end
      |     if (imax<=0)
      |       warning('Max. phase current must be positive.');
      |     end
      |     w0=6.283185307179586*wf0;
      |     pgain=2.0*wksi*w0*J/Kt;
      |     igain=w0*w0*J/Kt;
      |     fltPropGain=0.9*pgain;
      |     fltIntegGain=igain*SampleTime*0.5;
      |     if (Idmax<0)
      |       iratio=abs(Idmax)/imax;
      |       lowlim=acos(iratio)-1.570796326794897;
      |     else
      |       lowlim=0.0;
      |     end
      |     fltLowerLimit=lowlim;
      |     fltUpperLimit=0.0;
      |     fltLambda=lambdaFW;
      |     fltUmaxDivImax=0.5773502691896258*udcbus/imax;
      |     if isnan(fltUmaxDivImax)
      |       if ~strcmp(fltUmaxDivImax_bkup,'0')
      |         set_param(gcb,'fltUmaxDivImax','0');
      |       end
      |     else
      |       tmps=num2str(fltUmaxDivImax);
      |       if ~strcmp(fltUmaxDivImax_bkup,tmps)
      |         set_param(gcb,'fltUmaxDivImax',tmps);
      |       end
      |     end
      |     if isnan(fltLambda)
      |       if ~strcmp(fltLambda_bkup,'0')
      |         set_param(gcb,'fltLambda','0');
      |       end
      |     else
      |       tmps=num2str(fltLambda);
      |       if ~strcmp(fltLambda_bkup,tmps)
      |         set_param(gcb,'fltLambda',tmps);
      |       end
      |     end
      |     if isnan(fltPropGain)
      |       if ~strcmp(fltPropGain_bkup,'0')
      |         set_param(gcb,'fltPropGain','0');
      |       end
      |     else
      |       tmps=num2str(fltPropGain);
      |       if ~strcmp(fltPropGain_bkup,tmps)
      |         set_param(gcb,'fltPropGain',tmps);
      |       end
      |     end
      |     if isnan(fltIntegGain)
      |       if ~strcmp(fltIntegGain_bkup,'0')
      |         set_param(gcb,'fltIntegGain','0');
      |       end
      |     else
      |       tmps=num2str(fltIntegGain);
      |       if ~strcmp(fltIntegGain_bkup,tmps)
      |         set_param(gcb,'fltIntegGain',tmps);
      |       end
      |     end
      |     if isnan(fltLowerLimit)
      |       if ~strcmp(fltLowerLimit_bkup,'0')
      |         set_param(gcb,'fltLowerLimit','0');
      |       end
      |     else
      |       tmps=num2str(fltLowerLimit);
      |       if ~strcmp(fltLowerLimit_bkup,tmps)
      |         set_param(gcb,'fltLowerLimit',tmps);
      |       end
      |     end
      |     if isnan(fltUpperLimit)
      |       if ~strcmp(fltUpperLimit_bkup,'0')
      |         set_param(gcb,'fltUpperLimit','0');
      |       end
      |     else
      |       tmps=num2str(fltUpperLimit);
      |       if ~strcmp(fltUpperLimit_bkup,tmps)
      |         set_param(gcb,'fltUpperLimit',tmps);
      |       end
      |     end
      |   else
      |     param=p.getParameter('udcbus');
      |     if strcmp(param.Enabled,'on')
      |       hintText.Prompt='Caution: Implementation parameters are fixed.';
      |       p=Simulink.Mask.get(gcb);
      |       param=p.getParameter('wf0');
      |       param.set('Enabled','off');
      |       param=p.getParameter('wksi');
      |       param.set('Enabled','off');
      |       param=p.getParameter('J');
      |       param.set('Enabled','off');
      |       param=p.getParameter('Kt');
      |       param.set('Enabled','off');
      |       param=p.getParameter('lambdaFW');
      |       param.set('Enabled','off');
      |       param=p.getParameter('Idmax');
      |       param.set('Enabled','off');
      |       param=p.getParameter('imax');
      |       param.set('Enabled','off');
      |       param=p.getParameter('udcbus');
      |       param.set('Enabled','off');
      |     end
      |   end
      | end
      mask DialogControl CompBut Prompt: Recalculate sample times
      mask DialogControl CompBut Tooltip: Simulink updates the sample times of all blocks when the simulation is run. This button will update the sample times now.
      mask DialogControl CompBut Callback:
      | btn=questdlg('This will apply all changes in all open dialog boxes and update the schematic. Do you want to proceed?','Apply all changes','Continue','Cancel','Continue');
      | if strcmp(btn,'Continue')
      |   dlgs=DAStudio.ToolRoot.getOpenDialogs;
      |   for i=1:length(dlgs)
      |     dlgs(i).apply;
      |   end
      |   try
      |     SampleTime_1=str2double(get_param(gcb,'SampleTime_1'));
      |     ts=Simulink.Block.getSampleTimes(gcb);
      |     ts=ts(1).Value(1);
      |     if (SampleTime_1 ~= ts)
      |       SampleTime_1=ts;
      |       set_param(gcb,'SampleTime_1',num2str(ts));
      |       autoCalcEn=get_param(gcb,'autoCalcEn');
      |       if strcmp(autoCalcEn,'on')
      |         SampleTime=Simulink.data.evalinGlobal(bdroot,get_param(gcb,'SampleTime'));
      |         p=Simulink.Mask.get(gcb);
      |         hintText=p.getDialogControl('timeHint');
      |         if SampleTime==-1
      |           SampleTime=SampleTime_1;
      |           hintText.Prompt='Caution: Implementation parameters depend on inherited sample time. Make sure that the sample time of the block''s inputs corresponds to the sampling period in the target application.';
      |         else
      |           hintText.Prompt='Caution: Implementation parameters depend on the sample time. Make sure that the simulation time step corresponds to the sampling period in the target application.';
      |         end
      |         fltUmaxDivImax_bkup=get_param(gcb,'fltUmaxDivImax');
      |         fltLambda_bkup=get_param(gcb,'fltLambda');
      |         fltPropGain_bkup=get_param(gcb,'fltPropGain');
      |         fltIntegGain_bkup=get_param(gcb,'fltIntegGain');
      |         fltLowerLimit_bkup=get_param(gcb,'fltLowerLimit');
      |         fltUpperLimit_bkup=get_param(gcb,'fltUpperLimit');
      |         wf0=Simulink.data.evalinGlobal(bdroot,get_param(gcb,'wf0'));
      |         wksi=Simulink.data.evalinGlobal(bdroot,get_param(gcb,'wksi'));
      |         J=Simulink.data.evalinGlobal(bdroot,get_param(gcb,'J'));
      |         Kt=Simulink.data.evalinGlobal(bdroot,get_param(gcb,'Kt'));
      |         lambdaFW=Simulink.data.evalinGlobal(bdroot,get_param(gcb,'lambdaFW'));
      |         Idmax=Simulink.data.evalinGlobal(bdroot,get_param(gcb,'Idmax'));
      |         imax=Simulink.data.evalinGlobal(bdroot,get_param(gcb,'imax'));
      |         udcbus=Simulink.data.evalinGlobal(bdroot,get_param(gcb,'udcbus'));
      |         if (wf0<=0)
      |           warning('Natural frequency f0 must be positive.');
      |         end
      |         if (wksi<=0)
      |           warning('Current loop attenuation must be positive.');
      |         end
      |         if (wksi>1)
      |           warning('Current loop attenuation must not exceed 1.');
      |         end
      |         if (J<=0)
      |           warning('Moment of inertia J must be positive.');
      |         end
      |         if (Kt<=0)
      |           warning('Torque constant Kt must be positive.');
      |         end
      |         if (lambdaFW<0)
      |           warning('MA filter smoothing factor must be in the range 0..1.');
      |         end
      |         if (lambdaFW>1)
      |           warning('MA filter smoothing factor must be in the range 0..1.');
      |         end
      |         if (udcbus<=0)
      |           warning('DC bus voltage must be positive.');
      |         end
      |         if (imax<=0)
      |           warning('Max. phase current must be positive.');
      |         end
      |         w0=6.283185307179586*wf0;
      |         pgain=2.0*wksi*w0*J/Kt;
      |         igain=w0*w0*J/Kt;
      |         fltPropGain=0.9*pgain;
      |         fltIntegGain=igain*SampleTime*0.5;
      |         if (Idmax<0)
      |           iratio=abs(Idmax)/imax;
      |           lowlim=acos(iratio)-1.570796326794897;
      |         else
      |           lowlim=0.0;
      |         end
      |         fltLowerLimit=lowlim;
      |         fltUpperLimit=0.0;
      |         fltLambda=lambdaFW;
      |         fltUmaxDivImax=0.5773502691896258*udcbus/imax;
      |         if isnan(fltUmaxDivImax)
      |           if ~strcmp(fltUmaxDivImax_bkup,'0')
      |             set_param(gcb,'fltUmaxDivImax','0');
      |           end
      |         else
      |           tmps=num2str(fltUmaxDivImax);
      |           if ~strcmp(fltUmaxDivImax_bkup,tmps)
      |             set_param(gcb,'fltUmaxDivImax',tmps);
      |           end
      |         end
      |         if isnan(fltLambda)
      |           if ~strcmp(fltLambda_bkup,'0')
      |             set_param(gcb,'fltLambda','0');
      |           end
      |         else
      |           tmps=num2str(fltLambda);
      |           if ~strcmp(fltLambda_bkup,tmps)
      |             set_param(gcb,'fltLambda',tmps);
      |           end
      |         end
      |         if isnan(fltPropGain)
      |           if ~strcmp(fltPropGain_bkup,'0')
      |             set_param(gcb,'fltPropGain','0');
      |           end
      |         else
      |           tmps=num2str(fltPropGain);
      |           if ~strcmp(fltPropGain_bkup,tmps)
      |             set_param(gcb,'fltPropGain',tmps);
      |           end
      |         end
      |         if isnan(fltIntegGain)
      |           if ~strcmp(fltIntegGain_bkup,'0')
      |             set_param(gcb,'fltIntegGain','0');
      |           end
      |         else
      |           tmps=num2str(fltIntegGain);
      |           if ~strcmp(fltIntegGain_bkup,tmps)
      |             set_param(gcb,'fltIntegGain',tmps);
      |           end
      |         end
      |         if isnan(fltLowerLimit)
      |           if ~strcmp(fltLowerLimit_bkup,'0')
      |             set_param(gcb,'fltLowerLimit','0');
      |           end
      |         else
      |           tmps=num2str(fltLowerLimit);
      |           if ~strcmp(fltLowerLimit_bkup,tmps)
      |             set_param(gcb,'fltLowerLimit',tmps);
      |           end
      |         end
      |         if isnan(fltUpperLimit)
      |           if ~strcmp(fltUpperLimit_bkup,'0')
      |             set_param(gcb,'fltUpperLimit','0');
      |           end
      |         else
      |           tmps=num2str(fltUpperLimit);
      |           if ~strcmp(fltUpperLimit_bkup,tmps)
      |             set_param(gcb,'fltUpperLimit',tmps);
      |           end
      |         end
      |       end
      |     end
      |   catch
      |    warning(['Sample time cannot be calculated for the block ' gcb])
      |   end
      | end
      mask DialogControl timeHint Prompt: Note: Implementation parameters cannot be calculated yet because the block's inherited sample time is unknown. Simulink will update the sample time when you run the simulation.
      mask Display:
      | color('black');
      | pos = get_param(gcb, 'Position');
      | width = pos(3) - pos(1);
      | height = pos(4) - pos(2);
      | tX=width/2;
      | tY=height - 25;
      | color('black');
      | text(tX,tY, 'AMCLIB_FW_FLT', 'horizontalAlignment', 'center');
      | if showStates == 2
      |   color('red');
      |   text(tX,tY - 20, ['debugging mode' char(13) char(10) '(limited performance)'], 'horizontalAlignment', 'center');
      | end
  AMCLIB_FluxEstimAB_FLT : Subsystem  TreatAsAtomicUnit=on  mask(AMCLIB_FluxEstimAB_FLT){showStates=Hide (faster execution), fltRs=0.33, fltLs=6e-4}
      mask prompts: showStates "Show parameters as inputs:"; fltRs "Winding resistance fltRs [Ohm]"; fltLs "Stator inductance fltLs [H]"
      mask help: This block calculates the PMSM rotor position by estimating the rotor flux in the Alpha-Beta reference frame. The function can be used for sensorless FOC in single precision floating-point implementation.
      mask init:
      | ddName = get_param(bdroot,'DataDictionary');
      | if length(ddName)==0
      |   set_param(bdroot,'DataDictionary','ammclib_types.sldd');
      | else
      |   dd = Simulink.data.dictionary.open(ddName);
      |   data = getSection(dd,'Design Data');
      |   if ~exist(data,'SWLIBS_2Syst_F16')
      |     addDataSource(dd,'ammclib_types.sldd');
      |     saveChanges(dd);
      |   end
      | end
      | 
      | if showStates == 1
      |   % hidden state variables
      |   if strcmp(get_param([gcb '/fltRs'], 'BlockType'), 'Inport')
      |     posblk = get_param(gcb, 'Position');
      | 
      |     pos = get_param([gcb, '/fltRs'], 'Position');
      |     orient = get_param([gcb, '/fltRs'], 'Orientation');
      |     delete_block([gcb, '/fltRs']);
      |     add_block('built-in/Ground', [gcb, '/fltRs'], 'Position', pos, 'Orientation', orient);
      | 
      |     pos = get_param([gcb, '/fltLs'], 'Position');
      |     orient = get_param([gcb, '/fltLs'], 'Orientation');
      |     delete_block([gcb, '/fltLs']);
      |     add_block('built-in/Ground', [gcb, '/fltLs'], 'Position', pos, 'Orientation', orient);
      | 
      | 
      |     set_param([gcb '/fltVelocity'], 'Port', '1');
      |     set_param([gcb '/pIAB'], 'Port', '2');
      |     set_param([gcb '/pUAB'], 'Port', '3');
      | 
      |     tmpOutCnt=0;
      |     tmpOutCnt=tmpOutCnt+1;
      |     set_param([gcb '/fltPhase'], 'Port', num2str(tmpOutCnt));
      | 
      | set_param(gcb,'MaskEnables',{'on','on','on'});
      | 
      |     if (posblk(4) - posblk(2)) > 100
      |       height = 100;
      |       set_param(gcb,'Position',[posblk(1), posblk(2), posblk(3), posblk(2)+height])
      |     end
      |   end
      | else
      |   % shown state variables
      |   if strcmp(get_param([gcb '/fltRs'], 'BlockType'), 'Ground')
      |     posblk = get_param(gcb, 'Position');
      | 
      |     pos = get_param([gcb, '/fltRs'], 'Position');
      |     orient = get_param([gcb, '/fltRs'], 'Orientation');
      |     delete_block([gcb, '/fltRs']);
      |     add_block('built-in/Inport', [gcb, '/fltRs'], 'Position', pos, 'Orientation', orient, 'OutDataTypeStr', 'single');
      | 
      |     pos = get_param([gcb, '/fltLs'], 'Position');
      |     orient = get_param([gcb, '/fltLs'], 'Orientation');
      |     delete_block([gcb, '/fltLs']);
      |     add_block('built-in/Inport', [gcb, '/fltLs'], 'Position', pos, 'Orientation', orient, 'OutDataTypeStr', 'single');
      | 
      | 
      | 
      | 
      |     set_param([gcb '/fltVelocity'], 'Port', '1');
      |     set_param([gcb '/pIAB'], 'Port', '2');
      |     set_param([gcb '/pUAB'], 'Port', '3');
      |     set_param([gcb '/fltRs'], 'Port', '4');
      |     set_param([gcb '/fltLs'], 'Port', '5');
      | 
      |     tmpOutCnt=0;
      |     tmpOutCnt=tmpOutCnt+1;
      |     set_param([gcb '/fltPhase'], 'Port', num2str(tmpOutCnt));
      | 
      |     set_param(gcb,'MaskEnables',{'on','off','off'});
      | 
      |     if (posblk(4) - posblk(2)) < 150
      |       height = 150;
      |       set_param(gcb,'Position',[posblk(1), posblk(2), posblk(3), posblk(2)+height])
      |     end
      |   end
      | end
      settings: RTWSystemCode=Inline
      mask Help: web([fileparts(which('ammclib_bam_S32K3xx.slx')) '/../doc/S32K3XXMCLUG.pdf'], '-browser')
      mask TypeOptions showStates: Hide (faster execution) | Show (parameters can be changed during simulation)
      mask Callback showStates:
      | maskStr=get_param(gcb,'showStates');
      | if strcmp(maskStr,'Hide (faster execution)')
      |   if strcmp(get_param([gcb '/fltRs'], 'BlockType'), 'Inport')
      | set_param(gcb,'MaskEnables',{'on','on','on'});
      |   end
      | else
      |   if strcmp(get_param([gcb '/fltRs'], 'BlockType'), 'Ground')
      |     set_param(gcb,'MaskEnables',{'on','off','off'});
      |   end
      | end
      mask Display:
      | color('black');
      | pos = get_param(gcb, 'Position');
      | width = pos(3) - pos(1);
      | height = pos(4) - pos(2);
      | tX=width/2;
      | tY=height - 8;
      | color('black');
